simulink model "COMPONENT_MDL_Lag_QUAD_and_PEND_with_spin_rotors"  (R2021b)
settings: Solver=ode23t  StartTime=0.0  StopTime=200  FixedStep=0.001  RelTol=1e-5  EnableMultiTasking=on
undefined symbols (not defined in the file or in its folder): P_pend, P_rot, P_veh_no_props
(part 7 of 10)

== matlab function COMPONENT_MDL_Lag_QUAD_and_PEND_with_spin_rotors/bh_6DOF_and_pend/BUP/MCKGQ ==
  data: I_xx input; M output; I_xy input; I_xz input; I_yy input; I_yz input; I_zz input; Iprop_xx input; Iprop_xy input; Iprop_xz input; Iprop_yy input; Iprop_yz input; Iprop_zz input; Lx_pend input; Ly_pend input; Lz_pend input; Mbz_1 input; Mbz_2 input; Mbz_3 input; Mbz_4 input; THE_Phi input; THE_Psi input; THE_Phi_D input; THE_Psi_D input; THE_Theta input; THE_Theta_D input; THE_Phi_pend input; THE_Psi_pend input; THE_Phi_pend_D input; THE_Psi_pend_D input; THE_Theta_pend input; THE_Theta_pend_D input; Tbz_1 input; Tbz_2 input; Tbz_3 input; Tbz_4 input; Tv_Z_pend input; cg_to_mot_H input; cg_to_mot_L input; g input; m input; m_pend input; mprop input; wMOT_1 input; wMOT_2 input; wMOT_3 input; wMOT_4 input; C output; K output; G output; Q output
function [M,C,K,G,Q] = MCKGQ(I_xx,I_xy,I_xz,I_yy,I_yz,I_zz,Iprop_xx,Iprop_xy,Iprop_xz,Iprop_yy,Iprop_yz,Iprop_zz,Lx_pend,Ly_pend,Lz_pend,Mbz_1,Mbz_2,Mbz_3,Mbz_4,THE_Phi,THE_Psi,THE_Phi_D,THE_Psi_D,THE_Theta,THE_Theta_D,THE_Phi_pend,THE_Psi_pend,THE_Phi_pend_D,THE_Psi_pend_D,THE_Theta_pend,THE_Theta_pend_D,Tbz_1,Tbz_2,Tbz_3,Tbz_4,Tv_Z_pend,cg_to_mot_H,cg_to_mot_L,g,m,m_pend,mprop,wMOT_1,wMOT_2,wMOT_3,wMOT_4)
%#codegen

%    This function was generated by the Symbolic Math Toolbox version 8.6.
%    21-Sep-2020 14:08:37

M = reshape([I_xx+Iprop_xx.*4.0+(Lx_pend.^2.*m_pend)./1.2e+1+(Ly_pend.^2.*m_pend)./1.2e+1+Tv_Z_pend.^2.*m_pend+cg_to_mot_H.^2.*mprop.*4.0+cg_to_mot_L.^2.*mprop.*2.0-I_xx.*cos(THE_Theta).^2+I_yy.*cos(THE_Theta).^2-Iprop_xx.*cos(THE_Theta).^2.*4.0+Iprop_yy.*cos(THE_Theta).^2.*4.0-(Ly_pend.^2.*m_pend.*cos(THE_Theta).^2)./1.2e+1-(Ly_pend.^2.*m_pend.*cos(THE_Phi_pend).^2)./1.2e+1-(Ly_pend.^2.*m_pend.*cos(THE_Psi_pend).^2)./1.2e+1+(Lz_pend.^2.*m_pend.*cos(THE_Theta).^2)./3.0+(Lz_pend.^2.*m_pend.*cos(THE_Phi_pend).^2)./3.0+(Lz_pend.^2.*m_pend.*cos(THE_Psi_pend).^2)./3.0-I_yy.*cos(THE_Psi).^2.*cos(THE_Theta).^2+I_zz.*cos(THE_Psi).^2.*cos(THE_Theta).^2-Iprop_yy.*cos(THE_Psi).^2.*cos(THE_Theta).^2.*4.0+Iprop_zz.*cos(THE_Psi).^2.*cos(THE_Theta).^2.*4.0+I_yz.*cos(THE_Psi).*cos(THE_Theta).^2.*sin(THE_Psi).*2.0+Iprop_yz.*cos(THE_Psi).*cos(THE_Theta).^2.*sin(THE_Psi).*8.0-(Lx_pend.^2.*m_pend.*cos(THE_Psi).^2.*cos(THE_Theta).^2)./1.2e+1-(Lx_pend.^2.*m_pend.*cos(THE_Theta).^2.*cos(THE_Theta_pend).^2)./1.2e+1-(Lx_pend.^2.*m_pend.*cos(THE_Phi_pend).^2.*cos(THE_Theta_pend).^2)./1.2e+1+(Ly_pend.^2.*m_pend.*cos(THE_Psi).^2.*cos(THE_Theta).^2)./1.2e+1+(Ly_pend.^2.*m_pend.*cos(THE_Theta).^2.*cos(THE_Phi_pend).^2)./6.0+(Ly_pend.^2.*m_pend.*cos(THE_Theta).^2.*cos(THE_Psi_pend).^2)./6.0+(Ly_pend.^2.*m_pend.*cos(THE_Theta).^2.*cos(THE_Theta_pend).^2)./1.2e+1+(Ly_pend.^2.*m_pend.*cos(THE_Phi_pend).^2.*cos(THE_Psi_pend).^2)./6.0+(Ly_pend.^2.*m_pend.*cos(THE_Phi_pend).^2.*cos(THE_Theta_pend).^2)./1.2e+1-Lz_pend.^2.*m_pend.*cos(THE_Theta).^2.*cos(THE_Phi_pend).^2.*(2.0./3.0)-Lz_pend.^2.*m_pend.*cos(THE_Theta).^2.*cos(THE_Psi_pend).^2.*(2.0./3.0)-Lz_pend.^2.*m_pend.*cos(THE_Phi_pend).^2.*cos(THE_Psi_pend).^2.*(2.0./3.0)-Tv_Z_pend.^2.*m_pend.*cos(THE_Psi).^2.*cos(THE_Theta).^2-cg_to_mot_H.^2.*mprop.*cos(THE_Psi).^2.*cos(THE_Theta).^2.*4.0+cg_to_mot_L.^2.*mprop.*cos(THE_Psi).^2.*cos(THE_Theta).^2.*2.0-I_xz.*cos(THE_Psi).*cos(THE_Theta).*sin(THE_Theta).*2.0-Iprop_xz.*cos(THE_Psi).*cos(THE_Theta).*sin(THE_Theta).*8.0-I_xy.*cos(THE_Theta).*sin(THE_Psi).*sin(THE_Theta).*2.0-Iprop_xy.*cos(THE_Theta).*sin(THE_Psi).*sin(THE_Theta).*8.0+(Lx_pend.^2.*m_pend.*cos(THE_Psi).^2.*cos(THE_Theta).^2.*cos(THE_Theta_pend).^2)./6.0+(Lx_pend.^2.*m_pend.*cos(THE_Theta).^2.*cos(THE_Phi_pend).^2.*cos(THE_Theta_pend).^2)./6.0-(Ly_pend.^2.*m_pend.*cos(THE_Psi).^2.*cos(THE_Theta).^2.*cos(THE_Phi_pend).^2)./1.2e+1-(Ly_pend.^2.*m_pend.*cos(THE_Psi).^2.*cos(THE_Theta).^2.*cos(THE_Psi_pend).^2)./1.2e+1-(Ly_pend.^2.*m_pend.*cos(THE_Psi).^2.*cos(THE_Theta).^2.*cos(THE_Theta_pend).^2)./6.0-(Ly_pend.^2.*m_pend.*cos(THE_Theta).^2.*cos(THE_Phi_pend).^2.*cos(THE_Psi_pend).^2)./3.0-(Ly_pend.^2.*m_pend.*cos(THE_Theta).^2.*cos(THE_Phi_pend).^2.*cos(THE_Theta_pend).^2)./6.0-(Ly_pend.^2.*m_pend.*cos(THE_Theta).^2.*cos(THE_Psi_pend).^2.*cos(THE_Theta_pend).^2)./1.2e+1-(Ly_pend.^2.*m_pend.*cos(THE_Phi_pend).^2.*cos(THE_Psi_pend).^2.*cos(THE_Theta_pend).^2)./1.2e+1+(Lz_pend.^2.*m_pend.*cos(THE_Psi).^2.*cos(THE_Theta).^2.*cos(THE_Phi_pend).^2)./3.0+(Lz_pend.^2.*m_pend.*cos(THE_Psi).^2.*cos(THE_Theta).^2.*cos(THE_Psi_pend).^2)./3.0+Lz_pend.^2.*m_pend.*cos(THE_Theta).^2.*cos(THE_Phi_pend).^2.*cos(THE_Psi_pend).^2.*(4.0./3.0)+(Lz_pend.^2.*m_pend.*cos(THE_Theta).^2.*cos(THE_Psi_pend).^2.*cos(THE_Theta_pend).^2)./3.0+(Lz_pend.^2.*m_pend.*cos(THE_Phi_pend).^2.*cos(THE_Psi_pend).^2.*cos(THE_Theta_pend).^2)./3.0+Lz_pend.*Tv_Z_pend.*m_pend.*cos(THE_Psi_pend).*cos(THE_Theta_pend)-(Lx_pend.^2.*m_pend.*cos(THE_Psi).^2.*cos(THE_Theta).^2.*cos(THE_Phi_pend).^2.*cos(THE_Theta_pend).^2)./1.2e+1+(Ly_pend.^2.*m_pend.*cos(THE_Psi).^2.*cos(THE_Theta).^2.*cos(THE_Phi_pend).^2.*cos(THE_Psi_pend).^2)./6.0+(Ly_pend.^2.*m_pend.*cos(THE_Psi).^2.*cos(THE_Theta).^2.*cos(THE_Phi_pend).^2.*cos(THE_Theta_pend).^2)./1.2e+1+(Ly_pend.^2.*m_pend.*cos(THE_Psi).^2.*cos(THE_Theta).^2.*cos(THE_Psi_pend).^2.*cos(THE_Theta_pend).^2)./6.0+(Ly_pend.^2.*m_pend.*cos(THE_Theta).^2.*cos(THE_Phi_pend).^2.*cos(THE_Psi_pend).^2.*cos(THE_Theta_pend).^2)./6.0-Lz_pend.^2.*m_pend.*cos(THE_Psi).^2.*cos(THE_Theta).^2.*cos(THE_Phi_pend).^2.*cos(THE_Psi_pend).^2.*(2.0./3.0)-Lz_pend.^2.*m_pend.*cos(THE_Psi).^2.*cos(THE_Theta).^2.*cos(THE_Psi_pend).^2.*cos(THE_Theta_pend).^2.*(2.0./3.0)-Lz_pend.^2.*m_pend.*cos(THE_Theta).^2.*cos(THE_Phi_pend).^2.*cos(THE_Psi_pend).^2.*cos(THE_Theta_pend).^2.*(2.0./3.0)-Lz_pend.*Tv_Z_pend.*m_pend.*cos(THE_Psi).^2.*cos(THE_Theta).^2.*cos(THE_Psi_pend).*cos(THE_Theta_pend)+(Ly_pend.^2.*m_pend.*cos(THE_Theta).*cos(THE_Phi_pend).*sin(THE_Psi).*sin(THE_Theta).*sin(THE_Phi_pend))./6.0+(Ly_pend.^2.*m_pend.*cos(THE_Phi_pend).*cos(THE_Psi_pend).*sin(THE_Phi_pend).*sin(THE_Psi_pend).*sin(THE_Theta_pend))./6.0-Lz_pend.^2.*m_pend.*cos(THE_Theta).*cos(THE_Phi_pend).*sin(THE_Psi).*sin(THE_Theta).*sin(THE_Phi_pend).*(2.0./3.0)-Lz_pend.^2.*m_pend.*cos(THE_Phi_pend).*cos(THE_Psi_pend).*sin(THE_Phi_pend).*sin(THE_Psi_pend).*sin(THE_Theta_pend).*(2.0./3.0)-(Ly_pend.^2.*m_pend.*cos(THE_Psi).^2.*cos(THE_Theta).^2.*cos(THE_Phi_pend).^2.*cos(THE_Psi_pend).^2.*cos(THE_Theta_pend).^2)./1.2e+1+(Lz_pend.^2.*m_pend.*cos(THE_Psi).^2.*cos(THE_Theta).^2.*cos(THE_Phi_pend).^2.*cos(THE_Psi_pend).^2.*cos(THE_Theta_pend).^2)./3.0-(Ly_pend.^2.*m_pend.*cos(THE_Theta).*cos(THE_Psi_pend).*sin(THE_Psi).*sin(THE_Theta).*sin(THE_Psi_pend).*sin(THE_Theta_pend))./6.0+Lz_pend.^2.*m_pend.*cos(THE_Theta).*cos(THE_Psi_pend).*sin(THE_Psi).*sin(THE_Theta).*sin(THE_Psi_pend).*sin(THE_Theta_pend).*(2.0./3.0)+Lz_pend.*Tv_Z_pend.*m_pend.*cos(THE_Psi).*cos(THE_Theta).*sin(THE_Theta).*sin(THE_Phi_pend).*sin(THE_Psi_pend)+(Lx_pend.^2.*m_pend.*cos(THE_Theta).*cos(THE_Phi_pend).*cos(THE_Theta_pend).^2.*sin(THE_Psi).*sin(THE_Theta).*sin(THE_Phi_pend))./6.0+(Lx_pend.^2.*m_pend.*cos(THE_Psi).*cos(THE_Theta).^2.*cos(THE_Theta_pend).*sin(THE_Psi).*sin(THE_Phi_pend).*sin(THE_Theta_pend))./6.0-(Ly_pend.^2.*m_pend.*cos(THE_Theta).*cos(THE_Phi_pend).*cos(THE_Psi_pend).^2.*sin(THE_Psi).*sin(THE_Theta).*sin(THE_Phi_pend))./3.0-(Ly_pend.^2.*m_pend.*cos(THE_Theta).*cos(THE_Phi_pend).*cos(THE_Theta_pend).^2.*sin(THE_Psi).*sin(THE_Theta).*sin(THE_Phi_pend))./6.0-(Ly_pend.^2.*m_pend.*cos(THE_Psi).*cos(THE_Theta).^2.*cos(THE_Theta_pend).*sin(THE_Psi).*sin(THE_Phi_pend).*sin(THE_Theta_pend))./6.0-(Ly_pend.^2.*m_pend.*cos(THE_Theta).^2.*cos(THE_Phi_pend).*cos(THE_Psi_pend).*sin(THE_Phi_pend).*sin(THE_Psi_pend).*sin(THE_Theta_pend))./3.0+Lz_pend.^2.*m_pend.*cos(THE_Theta).*cos(THE_Phi_pend).*cos(THE_Psi_pend).^2.*sin(THE_Psi).*sin(THE_Theta).*sin(THE_Phi_pend).*(4.0./3.0)+Lz_pend.^2.*m_pend.*cos(THE_Theta).^2.*cos(THE_Phi_pend).*cos(THE_Psi_pend).*sin(THE_Phi_pend).*sin(THE_Psi_pend).*sin(THE_Theta_pend).*(4.0./3.0)+Lz_pend.*Tv_Z_pend.*m_pend.*cos(THE_Psi).*cos(THE_Theta).^2.*cos(THE_Phi_pend).*sin(THE_Psi).*sin(THE_Psi_pend)-(Lx_pend.^2.*m_pend.*cos(THE_Psi).*cos(THE_Theta).*cos(THE_Phi_pend).*cos(THE_Theta_pend).*sin(THE_Theta).*sin(THE_Theta_pend))./6.0+(Ly_pend.^2.*m_pend.*cos(THE_Psi).*cos(THE_Theta).*cos(THE_Phi_pend).*cos(THE_Theta_pend).*sin(THE_Theta).*sin(THE_Theta_pend))./6.0+(Ly_pend.^2.*m_pend.*cos(THE_Theta).*cos(THE_Phi_pend).^2.*cos(THE_Psi_pend).*sin(THE_Psi).*sin(THE_Theta).*sin(THE_Psi_pend).*sin(THE_Theta_pend))./3.0-Lz_pend.^2.*m_pend.*cos(THE_Theta).*cos(THE_Phi_pend).^2.*cos(THE_Psi_pend).*sin(THE_Psi).*sin(THE_Theta).*sin(THE_Psi_pend).*sin(THE_Theta_pend).*(4.0./3.0)-Lz_pend.*Tv_Z_pend.*m_pend.*cos(THE_Psi).*cos(THE_Theta).^2.*cos(THE_Psi_pend).*sin(THE_Psi).*sin(THE_Phi_pend).*sin(THE_Theta_pend)+(Ly_pend.^2.*m_pend.*cos(THE_Theta).*cos(THE_Phi_pend).*cos(THE_Psi_pend).^2.*cos(THE_Theta_pend).^2.*sin(THE_Psi).*sin(THE_Theta).*sin(THE_Phi_pend))./6.0+(Ly_pend.^2.*m_pend.*cos(THE_Psi).*cos(THE_Theta).^2.*cos(THE_Psi_pend).^2.*cos(THE_Theta_pend).*sin(THE_Psi).*sin(THE_Phi_pend).*sin(THE_Theta_pend))./6.0+(Ly_pend.^2.*m_pend.*cos(THE_Psi).^2.*cos(THE_Theta).^2.*cos(THE_Phi_pend).*cos(THE_Psi_pend).*sin(THE_Phi_pend).*sin(THE_Psi_pend).*sin(THE_Theta_pend))./6.0-Lz_pend.^2.*m_pend.*cos(THE_Theta).*cos(THE_Phi_pend).*cos(THE_Psi_pend).^2.*cos(THE_Theta_pend).^2.*sin(THE_Psi).*sin(THE_Theta).*sin(THE_Phi_pend).*(2.0./3.0)-Lz_pend.^2.*m_pend.*cos(THE_Psi).*cos(THE_Theta).^2.*cos(THE_Psi_pend).^2.*cos(THE_Theta_pend).*sin(THE_Psi).*sin(THE_Phi_pend).*sin(THE_Theta_pend).*(2.0./3.0)-Lz_pend.^2.*m_pend.*cos(THE_Psi).^2.*cos(THE_Theta).^2.*cos(THE_Phi_pend).*cos(THE_Psi_pend).*sin(THE_Phi_pend).*sin(THE_Psi_pend).*sin(THE_Theta_pend).*(2.0./3.0)-(Ly_pend.^2.*m_pend.*cos(THE_Psi).*cos(THE_Theta).*cos(THE_Psi_pend).*cos(THE_Theta_pend).*sin(THE_Theta).*sin(THE_Phi_pend).*sin(THE_Psi_pend))./6.0+Lz_pend.^2.*m_pend.*cos(THE_Psi).*cos(THE_Theta).*cos(THE_Psi_pend).*cos(THE_Theta_pend).*sin(THE_Theta).*sin(THE_Phi_pend).*sin(THE_Psi_pend).*(2.0./3.0)+Lz_pend.*Tv_Z_pend.*m_pend.*cos(THE_Psi).*cos(THE_Theta).*cos(THE_Phi_pend).*cos(THE_Psi_pend).*sin(THE_Theta).*sin(THE_Theta_pend)-(Ly_pend.^2.*m_pend.*cos(THE_Psi).*cos(THE_Theta).^2.*cos(THE_Phi_pend).*cos(THE_Psi_pend).*cos(THE_Theta_pend).*sin(THE_Psi).*sin(THE_Psi_pend))./6.0-(Ly_pend.^2.*m_pend.*cos(THE_Psi).*cos(THE_Theta).*cos(THE_Phi_pend).*cos(THE_Psi_pend).^2.*cos(THE_Theta_pend).*sin(THE_Theta).*sin(THE_Theta_pend))./6.0+Lz_pend.^2.*m_pend.*cos(THE_Psi).*cos(THE_Theta).^2.*cos(THE_Phi_pend).*cos(THE_Psi_pend).*cos(THE_Theta_pend).*sin(THE_Psi).*sin(THE_Psi_pend).*(2.0./3.0)+Lz_pend.^2.*m_pend.*cos(THE_Psi).*cos(THE_Theta).*cos(THE_Phi_pend).*cos(THE_Psi_pend).^2.*cos(THE_Theta_pend).*sin(THE_Theta).*sin(THE_Theta_pend).*(2.0./3.0),-I_yz.*cos(THE_Theta)-Iprop_yz.*cos(THE_Theta).*4.0-I_xy.*cos(THE_Psi).*sin(THE_Theta)-Iprop_xy.*cos(THE_Psi).*sin(THE_Theta).*4.0+I_xz.*sin(THE_Psi).*sin(THE_Theta)+Iprop_xz.*sin(THE_Psi).*sin(THE_Theta).*4.0+I_yz.*cos(THE_Psi).^2.*cos(THE_Theta).*2.0+Iprop_yz.*cos(THE_Psi).^2.*cos(THE_Theta).*8.0+I_yy.*cos(THE_Psi).*cos(THE_Theta).*sin(THE_Psi)-I_zz.*cos(THE_Psi).*cos(THE_Theta).*sin(THE_Psi)+Iprop_yy.*cos(THE_Psi).*cos(THE_Theta).*sin(THE_Psi).*4.0-Iprop_zz.*cos(THE_Psi).*cos(THE_Theta).*sin(THE_Psi).*4.0+(Lx_pend.^2.*m_pend.*cos(THE_Psi).*cos(THE_Theta).*sin(THE_Psi))./1.2e+1-(Ly_pend.^2.*m_pend.*cos(THE_Psi).*cos(THE_Theta).*sin(THE_Psi))./1.2e+1+Tv_Z_pend.^2.*m_pend.*cos(THE_Psi).*cos(THE_Theta).*sin(THE_Psi)+cg_to_mot_H.^2.*mprop.*cos(THE_Psi).*cos(THE_Theta).*sin(THE_Psi).*4.0-cg_to_mot_L.^2.*mprop.*cos(THE_Psi).*cos(THE_Theta).*sin(THE_Psi).*2.0-(Lx_pend.^2.*m_pend.*cos(THE_Theta).*cos(THE_Theta_pend).*sin(THE_Phi_pend).*sin(THE_Theta_pend))./1.2e+1+(Ly_pend.^2.*m_pend.*cos(THE_Psi).*cos(THE_Phi_pend).*sin(THE_Theta).*sin(THE_Phi_pend))./1.2e+1+(Ly_pend.^2.*m_pend.*cos(THE_Theta).*cos(THE_Theta_pend).*sin(THE_Phi_pend).*sin(THE_Theta_pend))./1.2e+1-(Lz_pend.^2.*m_pend.*cos(THE_Psi).*cos(THE_Phi_pend).*sin(THE_Theta).*sin(THE_Phi_pend))./3.0-(Lz_pend.*Tv_Z_pend.*m_pend.*cos(THE_Theta).*cos(THE_Phi_pend).*sin(THE_Psi_pend))./2.0-(Lx_pend.^2.*m_pend.*cos(THE_Psi).*cos(THE_Theta).*cos(THE_Theta_pend).^2.*sin(THE_Psi))./6.0+(Ly_pend.^2.*m_pend.*cos(THE_Psi).*cos(THE_Theta).*cos(THE_Phi_pend).^2.*sin(THE_Psi))./1.2e+1+(Ly_pend.^2.*m_pend.*cos(THE_Psi).*cos(THE_Theta).*cos(THE_Psi_pend).^2.*sin(THE_Psi))./1.2e+1+(Ly_pend.^2.*m_pend.*cos(THE_Psi).*cos(THE_Theta).*cos(THE_Theta_pend).^2.*sin(THE_Psi))./6.0-(Lz_pend.^2.*m_pend.*cos(THE_Psi).*cos(THE_Theta).*cos(THE_Phi_pend).^2.*sin(THE_Psi))./3.0-(Lz_pend.^2.*m_pend.*cos(THE_Psi).*cos(THE_Theta).*cos(THE_Psi_pend).^2.*sin(THE_Psi))./3.0+(Ly_pend.^2.*m_pend.*cos(THE_Theta).*cos(THE_Phi_pend).*cos(THE_Psi_pend).*cos(THE_Theta_pend).*sin(THE_Psi_pend))./1.2e+1-(Lz_pend.^2.*m_pend.*cos(THE_Theta).*cos(THE_Phi_pend).*cos(THE_Psi_pend).*cos(THE_Theta_pend).*sin(THE_Psi_pend))./3.0+(Lx_pend.^2.*m_pend.*cos(THE_Phi_pend).*cos(THE_Theta_pend).*sin(THE_Psi).*sin(THE_Theta).*sin(THE_Theta_pend))./1.2e+1-(Ly_pend.^2.*m_pend.*cos(THE_Psi).*cos(THE_Psi_pend).*sin(THE_Theta).*sin(THE_Psi_pend).*sin(THE_Theta_pend))./1.2e+1-(Ly_pend.^2.*m_pend.*cos(THE_Phi_pend).*cos(THE_Theta_pend).*sin(THE_Psi).*sin(THE_Theta).*sin(THE_Theta_pend))./1.2e+1+(Lz_pend.^2.*m_pend.*cos(THE_Psi).*cos(THE_Psi_pend).*sin(THE_Theta).*sin(THE_Psi_pend).*sin(THE_Theta_pend))./3.0+(Lz_pend.*Tv_Z_pend.*m_pend.*cos(THE_Theta).*cos(THE_Psi_pend).*sin(THE_Phi_pend).*sin(THE_Theta_pend))./2.0-(Lz_pend.*Tv_Z_pend.*m_pend.*sin(THE_Psi).*sin(THE_Theta).*sin(THE_Phi_pend).*sin(THE_Psi_pend))./2.0+(Lx_pend.^2.*m_pend.*cos(THE_Psi).*cos(THE_Phi_pend).*cos(THE_Theta_pend).^2.*sin(THE_Theta).*sin(THE_Phi_pend))./1.2e+1+(Lx_pend.^2.*m_pend.*cos(THE_Psi).^2.*cos(THE_Theta).*cos(THE_Theta_pend).*sin(THE_Phi_pend).*sin(THE_Theta_pend))./6.0-(Ly_pend.^2.*m_pend.*cos(THE_Psi).*cos(THE_Phi_pend).*cos(THE_Psi_pend).^2.*sin(THE_Theta).*sin(THE_Phi_pend))./6.0-(Ly_pend.^2.*m_pend.*cos(THE_Psi).*cos(THE_Phi_pend).*cos(THE_Theta_pend).^2.*sin(THE_Theta).*sin(THE_Phi_pend))./1.2e+1-(Ly_pend.^2.*m_pend.*cos(THE_Psi).^2.*cos(THE_Theta).*cos(THE_Theta_pend).*sin(THE_Phi_pend).*sin(THE_Theta_pend))./6.0-(Ly_pend.^2.*m_pend.*cos(THE_Theta).*cos(THE_Psi_pend).^2.*cos(THE_Theta_pend).*sin(THE_Phi_pend).*sin(THE_Theta_pend))./1.2e+1+Lz_pend.^2.*m_pend.*cos(THE_Psi).*cos(THE_Phi_pend).*cos(THE_Psi_pend).^2.*sin(THE_Theta).*sin(THE_Phi_pend).*(2.0./3.0)+(Lz_pend.^2.*m_pend.*cos(THE_Theta).*cos(THE_Psi_pend).^2.*cos(THE_Theta_pend).*sin(THE_Phi_pend).*sin(THE_Theta_pend))./3.0+Lz_pend.*Tv_Z_pend.*m_pend.*cos(THE_Psi).^2.*cos(THE_Theta).*cos(THE_Phi_pend).*sin(THE_Psi_pend)+(Lx_pend.^2.*m_pend.*cos(THE_Psi).*cos(THE_Theta).*cos(THE_Phi_pend).^2.*cos(THE_Theta_pend).^2.*sin(THE_Psi))./1.2e+1-(Ly_pend.^2.*m_pend.*cos(THE_Psi).*cos(THE_Theta).*cos(THE_Phi_pend).^2.*cos(THE_Psi_pend).^2.*sin(THE_Psi))./6.0-(Ly_pend.^2.*m_pend.*cos(THE_Psi).*cos(THE_Theta).*cos(THE_Phi_pend).^2.*cos(THE_Theta_pend).^2.*sin(THE_Psi))./1.2e+1-(Ly_pend.^2.*m_pend.*cos(THE_Psi).*cos(THE_Theta).*cos(THE_Psi_pend).^2.*cos(THE_Theta_pend).^2.*sin(THE_Psi))./6.0+Lz_pend.^2.*m_pend.*cos(THE_Psi).*cos(THE_Theta).*cos(THE_Phi_pend).^2.*cos(THE_Psi_pend).^2.*sin(THE_Psi).*(2.0./3.0)+Lz_pend.^2.*m_pend.*cos(THE_Psi).*cos(THE_Theta).*cos(THE_Psi_pend).^2.*cos(THE_Theta_pend).^2.*sin(THE_Psi).*(2.0./3.0)+(Ly_pend.^2.*m_pend.*cos(THE_Psi_pend).*cos(THE_Theta_pend).*sin(THE_Psi).*sin(THE_Theta).*sin(THE_Phi_pend).*sin(THE_Psi_pend))./1.2e+1-(Lz_pend.^2.*m_pend.*cos(THE_Psi_pend).*cos(THE_Theta_pend).*sin(THE_Psi).*sin(THE_Theta).*sin(THE_Phi_pend).*sin(THE_Psi_pend))./3.0+Lz_pend.*Tv_Z_pend.*m_pend.*cos(THE_Psi).*cos(THE_Theta).*cos(THE_Psi_pend).*cos(THE_Theta_pend).*sin(THE_Psi)-(Lz_pend.*Tv_Z_pend.*m_pend.*cos(THE_Phi_pend).*cos(THE_Psi_pend).*sin(THE_Psi).*sin(THE_Theta).*sin(THE_Theta_pend))./2.0-(Ly_pend.^2.*m_pend.*cos(THE_Psi).^2.*cos(THE_Theta).*cos(THE_Phi_pend).*cos(THE_Psi_pend).*cos(THE_Theta_pend).*sin(THE_Psi_pend))./6.0+Lz_pend.^2.*m_pend.*cos(THE_Psi).^2.*cos(THE_Theta).*cos(THE_Phi_pend).*cos(THE_Psi_pend).*cos(THE_Theta_pend).*sin(THE_Psi_pend).*(2.0./3.0)+(Ly_pend.^2.*m_pend.*cos(THE_Psi).*cos(THE_Phi_pend).^2.*cos(THE_Psi_pend).*sin(THE_Theta).*sin(THE_Psi_pend).*sin(THE_Theta_pend))./6.0+(Ly_pend.^2.*m_pend.*cos(THE_Phi_pend).*cos(THE_Psi_pend).^2.*cos(THE_Theta_pend).*sin(THE_Psi).*sin(THE_Theta).*sin(THE_Theta_pend))./1.2e+1-Lz_pend.^2.*m_pend.*cos(THE_Psi).*cos(THE_Phi_pend).^2.*cos(THE_Psi_pend).*sin(THE_Theta).*sin(THE_Psi_pend).*sin(THE_Theta_pend).*(2.0./3.0)-(Lz_pend.^2.*m_pend.*cos(THE_Phi_pend).*cos(THE_Psi_pend).^2.*cos(THE_Theta_pend).*sin(THE_Psi).*sin(THE_Theta).*sin(THE_Theta_pend))./3.0-Lz_pend.*Tv_Z_pend.*m_pend.*cos(THE_Psi).^2.*cos(THE_Theta).*cos(THE_Psi_pend).*sin(THE_Phi_pend).*sin(THE_Theta_pend)+(Ly_pend.^2.*m_pend.*cos(THE_Psi).*cos(THE_Phi_pend).*cos(THE_Psi_pend).^2.*cos(THE_Theta_pend).^2.*sin(THE_Theta).*sin(THE_Phi_pend))./1.2e+1+(Ly_pend.^2.*m_pend.*cos(THE_Psi).^2.*cos(THE_Theta).*cos(THE_Psi_pend).^2.*cos(THE_Theta_pend).*sin(THE_Phi_pend).*sin(THE_Theta_pend))./6.0-(Lz_pend.^2.*m_pend.*cos(THE_Psi).*cos(THE_Phi_pend).*cos(THE_Psi_pend).^2.*cos(THE_Theta_pend).^2.*sin(THE_Theta).*sin(THE_Phi_pend))./3.0-Lz_pend.^2.*m_pend.*cos(THE_Psi).^2.*cos(THE_Theta).*cos(THE_Psi_pend).^2.*cos(THE_Theta_pend).*sin(THE_Phi_pend).*sin(THE_Theta_pend).*(2.0./3.0)+(Ly_pend.^2.*m_pend.*cos(THE_Psi).*cos(THE_Theta).*cos(THE_Phi_pend).^2.*cos(THE_Psi_pend).^2.*cos(THE_Theta_pend).^2.*sin(THE_Psi))./1.2e+1-(Lz_pend.^2.*m_pend.*cos(THE_Psi).*cos(THE_Theta).*cos(THE_Phi_pend).^2.*cos(THE_Psi_pend).^2.*cos(THE_Theta_pend).^2.*sin(THE_Psi))./3.0-(Ly_pend.^2.*m_pend.*cos(THE_Psi).*cos(THE_Theta).*cos(THE_Phi_pend).*cos(THE_Psi_pend).*sin(THE_Psi).*sin(THE_Phi_pend).*sin(THE_Psi_pend).*sin(THE_Theta_pend))./6.0+Lz_pend.^2.*m_pend.*cos(THE_Psi).*cos(THE_Theta).*cos(THE_Phi_pend).*cos(THE_Psi_pend).*sin(THE_Psi).*sin(THE_Phi_pend).*sin(THE_Psi_pend).*sin(THE_Theta_pend).*(2.0./3.0),-I_xx.*sin(THE_Theta)-Iprop_xx.*sin(THE_Theta).*4.0+I_xz.*cos(THE_Psi).*cos(THE_Theta)+Iprop_xz.*cos(THE_Psi).*cos(THE_Theta).*4.0+I_xy.*cos(THE_Theta).*sin(THE_Psi)+Iprop_xy.*cos(THE_Theta).*sin(THE_Psi).*4.0-(Lx_pend.^2.*m_pend.*sin(THE_Theta))./1.2e+1-(Ly_pend.^2.*m_pend.*sin(THE_Theta))./1.2e+1-Tv_Z_pend.^2.*m_pend.*sin(THE_Theta)-cg_to_mot_H.^2.*mprop.*sin(THE_Theta).*4.0-cg_to_mot_L.^2.*mprop.*sin(THE_Theta).*2.0+(Ly_pend.^2.*m_pend.*cos(THE_Phi_pend).^2.*sin(THE_Theta))./1.2e+1+(Ly_pend.^2.*m_pend.*cos(THE_Psi_pend).^2.*sin(THE_Theta))./1.2e+1-(Lz_pend.^2.*m_pend.*cos(THE_Phi_pend).^2.*sin(THE_Theta))./3.0-(Lz_pend.^2.*m_pend.*cos(THE_Psi_pend).^2.*sin(THE_Theta))./3.0+(Lx_pend.^2.*m_pend.*cos(THE_Phi_pend).^2.*cos(THE_Theta_pend).^2.*sin(THE_Theta))./1.2e+1-(Ly_pend.^2.*m_pend.*cos(THE_Phi_pend).^2.*cos(THE_Psi_pend).^2.*sin(THE_Theta))./6.0-(Ly_pend.^2.*m_pend.*cos(THE_Phi_pend).^2.*cos(THE_Theta_pend).^2.*sin(THE_Theta))./1.2e+1+Lz_pend.^2.*m_pend.*cos(THE_Phi_pend).^2.*cos(THE_Psi_pend).^2.*sin(THE_Theta).*(2.0./3.0)-(Ly_pend.^2.*m_pend.*cos(THE_Theta).*cos(THE_Phi_pend).*sin(THE_Psi).*sin(THE_Phi_pend))./1.2e+1+(Lz_pend.^2.*m_pend.*cos(THE_Theta).*cos(THE_Phi_pend).*sin(THE_Psi).*sin(THE_Phi_pend))./3.0+(Ly_pend.^2.*m_pend.*cos(THE_Phi_pend).^2.*cos(THE_Psi_pend).^2.*cos(THE_Theta_pend).^2.*sin(THE_Theta))./1.2e+1-(Lz_pend.^2.*m_pend.*cos(THE_Phi_pend).^2.*cos(THE_Psi_pend).^2.*cos(THE_Theta_pend).^2.*sin(THE_Theta))./3.0-Lz_pend.*Tv_Z_pend.*m_pend.*cos(THE_Psi_pend).*cos(THE_Theta_pend).*sin(THE_Theta)+(Lx_pend.^2.*m_pend.*cos(THE_Psi).*cos(THE_Theta).*cos(THE_Phi_pend).*cos(THE_Theta_pend).*sin(THE_Theta_pend))./1.2e+1-(Ly_pend.^2.*m_pend.*cos(THE_Psi).*cos(THE_Theta).*cos(THE_Phi_pend).*cos(THE_Theta_pend).*sin(THE_Theta_pend))./1.2e+1+(Ly_pend.^2.*m_pend.*cos(THE_Theta).*cos(THE_Psi_pend).*sin(THE_Psi).*sin(THE_Psi_pend).*sin(THE_Theta_pend))./1.2e+1-(Lz_pend.^2.*m_pend.*cos(THE_Theta).*cos(THE_Psi_pend).*sin(THE_Psi).*sin(THE_Psi_pend).*sin(THE_Theta_pend))./3.0-(Lz_pend.*Tv_Z_pend.*m_pend.*cos(THE_Psi).*cos(THE_Theta).*sin(THE_Phi_pend).*sin(THE_Psi_pend))./2.0-(Lx_pend.^2.*m_pend.*cos(THE_Theta).*cos(THE_Phi_pend).*cos(THE_Theta_pend).^2.*sin(THE_Psi).*sin(THE_Phi_pend))./1.2e+1+(Ly_pend.^2.*m_pend.*cos(THE_Theta).*cos(THE_Phi_pend).*cos(THE_Psi_pend).^2.*sin(THE_Psi).*sin(THE_Phi_pend))./6.0+(Ly_pend.^2.*m_pend.*cos(THE_Theta).*cos(THE_Phi_pend).*cos(THE_Theta_pend).^2.*sin(THE_Psi).*sin(THE_Phi_pend))./1.2e+1-Lz_pend.^2.*m_pend.*cos(THE_Theta).*cos(THE_Phi_pend).*cos(THE_Psi_pend).^2.*sin(THE_Psi).*sin(THE_Phi_pend).*(2.0./3.0)-(Ly_pend.^2.*m_pend.*cos(THE_Phi_pend).*cos(THE_Psi_pend).*sin(THE_Theta).*sin(THE_Phi_pend).*sin(THE_Psi_pend).*sin(THE_Theta_pend))./6.0+Lz_pend.^2.*m_pend.*cos(THE_Phi_pend).*cos(THE_Psi_pend).*sin(THE_Theta).*sin(THE_Phi_pend).*sin(THE_Psi_pend).*sin(THE_Theta_pend).*(2.0./3.0)-(Lz_pend.*Tv_Z_pend.*m_pend.*cos(THE_Psi).*cos(THE_Theta).*cos(THE_Phi_pend).*cos(THE_Psi_pend).*sin(THE_Theta_pend))./2.0+(Ly_pend.^2.*m_pend.*cos(THE_Psi).*cos(THE_Theta).*cos(THE_Phi_pend).*cos(THE_Psi_pend).^2.*cos(THE_Theta_pend).*sin(THE_Theta_pend))./1.2e+1-(Lz_pend.^2.*m_pend.*cos(THE_Psi).*cos(THE_Theta).*cos(THE_Phi_pend).*cos(THE_Psi_pend).^2.*cos(THE_Theta_pend).*sin(THE_Theta_pend))./3.0-(Ly_pend.^2.*m_pend.*cos(THE_Theta).*cos(THE_Phi_pend).^2.*cos(THE_Psi_pend).*sin(THE_Psi).*sin(THE_Psi_pend).*sin(THE_Theta_pend))./6.0+Lz_pend.^2.*m_pend.*cos(THE_Theta).*cos(THE_Phi_pend).^2.*cos(THE_Psi_pend).*sin(THE_Psi).*sin(THE_Psi_pend).*sin(THE_Theta_pend).*(2.0./3.0)-(Ly_pend.^2.*m_pend.*cos(THE_Theta).*cos(THE_Phi_pend).*cos(THE_Psi_pend).^2.*cos(THE_Theta_pend).^2.*sin(THE_Psi).*sin(THE_Phi_pend))./1.2e+1+(Lz_pend.^2.*m_pend.*cos(THE_Theta).*cos(THE_Phi_pend).*cos(THE_Psi_pend).^2.*cos(THE_Theta_pend).^2.*sin(THE_Psi).*sin(THE_Phi_pend))./3.0+(Ly_pend.^2.*m_pend.*cos(THE_Psi).*cos(THE_Theta).*cos(THE_Psi_pend).*cos(THE_Theta_pend).*sin(THE_Phi_pend).*sin(THE_Psi_pend))./1.2e+1-(Lz_pend.^2.*m_pend.*cos(THE_Psi).*cos(THE_Theta).*cos(THE_Psi_pend).*cos(THE_Theta_pend).*sin(THE_Phi_pend).*sin(THE_Psi_pend))./3.0,Tv_Z_pend.*m_pend.*cos(THE_Phi).*sin(THE_Psi)+cg_to_mot_H.*mprop.*cos(THE_Phi).*sin(THE_Psi).*4.0-Tv_Z_pend.*m_pend.*cos(THE_Psi).*sin(THE_Phi).*sin(THE_Theta)-cg_to_mot_H.*mprop.*cos(THE_Psi).*sin(THE_Phi).*sin(THE_Theta).*4.0+(Lz_pend.*m_pend.*cos(THE_Phi).*cos(THE_Psi).*cos(THE_Phi_pend).*sin(THE_Psi_pend))./2.0+(Lz_pend.*m_pend.*cos(THE_Phi).*cos(THE_Psi_pend).*cos(THE_Theta_pend).*sin(THE_Psi))./2.0-(Lz_pend.*m_pend.*cos(THE_Theta).*sin(THE_Phi).*sin(THE_Phi_pend).*sin(THE_Psi_pend))./2.0-(Lz_pend.*m_pend.*cos(THE_Psi).*cos(THE_Psi_pend).*cos(THE_Theta_pend).*sin(THE_Phi).*sin(THE_Theta))./2.0-(Lz_pend.*m_pend.*cos(THE_Phi).*cos(THE_Psi).*cos(THE_Psi_pend).*sin(THE_Phi_pend).*sin(THE_Theta_pend))./2.0-(Lz_pend.*m_pend.*cos(THE_Theta).*cos(THE_Phi_pend).*cos(THE_Psi_pend).*sin(THE_Phi).*sin(THE_Theta_pend))./2.0+(Lz_pend.*m_pend.*cos(THE_Phi_pend).*sin(THE_Phi).*sin(THE_Psi).*sin(THE_Theta).*sin(THE_Psi_pend))./2.0-(Lz_pend.*m_pend.*cos(THE_Psi_pend).*sin(THE_Phi).*sin(THE_Psi).*sin(THE_Theta).*sin(THE_Phi_pend).*sin(THE_Theta_pend))./2.0,Tv_Z_pend.*m_pend.*sin(THE_Phi).*sin(THE_Psi)+cg_to_mot_H.*mprop.*sin(THE_Phi).*sin(THE_Psi).*4.0+Tv_Z_pend.*m_pend.*cos(THE_Phi).*cos(THE_Psi).*sin(THE_Theta)+cg_to_mot_H.*mprop.*cos(THE_Phi).*cos(THE_Psi).*sin(THE_Theta).*4.0+(Lz_pend.*m_pend.*cos(THE_Psi).*cos(THE_Phi_pend).*sin(THE_Phi).*sin(THE_Psi_pend))./2.0+(Lz_pend.*m_pend.*cos(THE_Phi).*cos(THE_Theta).*sin(THE_Phi_pend).*sin(THE_Psi_pend))./2.0+(Lz_pend.*m_pend.*cos(THE_Psi_pend).*cos(THE_Theta_pend).*sin(THE_Phi).*sin(THE_Psi))./2.0+(Lz_pend.*m_pend.*cos(THE_Phi).*cos(THE_Psi).*cos(THE_Psi_pend).*cos(THE_Theta_pend).*sin(THE_Theta))./2.0+(Lz_pend.*m_pend.*cos(THE_Phi).*cos(THE_Theta).*cos(THE_Phi_pend).*cos(THE_Psi_pend).*sin(THE_Theta_pend))./2.0-(Lz_pend.*m_pend.*cos(THE_Phi).*cos(THE_Phi_pend).*sin(THE_Psi).*sin(THE_Theta).*sin(THE_Psi_pend))./2.0-(Lz_pend.*m_pend.*cos(THE_Psi).*cos(THE_Psi_pend).*sin(THE_Phi).*sin(THE_Phi_pend).*sin(THE_Theta_pend))./2.0+(Lz_pend.*m_pend.*cos(THE_Phi).*cos(THE_Psi_pend).*sin(THE_Psi).*sin(THE_Theta).*sin(THE_Phi_pend).*sin(THE_Theta_pend))./2.0,0.0,(Ly_pend.^2.*m_pend.*cos(THE_Psi).*cos(THE_Theta))./1.2e+1+(Lz_pend.^2.*m_pend.*cos(THE_Psi).*cos(THE_Theta))./3.0+(Lx_pend.^2.*m_pend.*cos(THE_Psi).*cos(THE_Theta).*cos(THE_Theta_pend).^2)./1.2e+1-(Ly_pend.^2.*m_pend.*cos(THE_Psi).*cos(THE_Theta).*cos(THE_Theta_pend).^2)./1.2e+1+(Ly_pend.^2.*m_pend.*cos(THE_Psi).*cos(THE_Theta).*cos(THE_Psi_pend).^2.*cos(THE_Theta_pend).^2)./1.2e+1-(Lz_pend.^2.*m_pend.*cos(THE_Psi).*cos(THE_Theta).*cos(THE_Psi_pend).^2.*cos(THE_Theta_pend).^2)./3.0-(Lx_pend.^2.*m_pend.*cos(THE_Phi_pend).*cos(THE_Theta_pend).*sin(THE_Theta).*sin(THE_Theta_pend))./1.2e+1+(Ly_pend.^2.*m_pend.*cos(THE_Phi_pend).*cos(THE_Theta_pend).*sin(THE_Theta).*sin(THE_Theta_pend))./1.2e+1+(Lz_pend.*Tv_Z_pend.*m_pend.*sin(THE_Theta).*sin(THE_Phi_pend).*sin(THE_Psi_pend))./2.0+(Lx_pend.^2.*m_pend.*cos(THE_Theta).*cos(THE_Theta_pend).*sin(THE_Psi).*sin(THE_Phi_pend).*sin(THE_Theta_pend))./1.2e+1-(Ly_pend.^2.*m_pend.*cos(THE_Theta).*cos(THE_Theta_pend).*sin(THE_Psi).*sin(THE_Phi_pend).*sin(THE_Theta_pend))./1.2e+1-(Ly_pend.^2.*m_pend.*cos(THE_Psi_pend).*cos(THE_Theta_pend).*sin(THE_Theta).*sin(THE_Phi_pend).*sin(THE_Psi_pend))./1.2e+1+(Lz_pend.^2.*m_pend.*cos(THE_Psi_pend).*cos(THE_Theta_pend).*sin(THE_Theta).*sin(THE_Phi_pend).*sin(THE_Psi_pend))./3.0+(Lz_pend.*Tv_Z_pend.*m_pend.*cos(THE_Theta).*cos(THE_Phi_pend).*sin(THE_Psi).*sin(THE_Psi_pend))./2.0+(Lz_pend.*Tv_Z_pend.*m_pend.*cos(THE_Phi_pend).*cos(THE_Psi_pend).*sin(THE_Theta).*sin(THE_Theta_pend))./2.0-(Ly_pend.^2.*m_pend.*cos(THE_Phi_pend).*cos(THE_Psi_pend).^2.*cos(THE_Theta_pend).*sin(THE_Theta).*sin(THE_Theta_pend))./1.2e+1+(Lz_pend.^2.*m_pend.*cos(THE_Phi_pend).*cos(THE_Psi_pend).^2.*cos(THE_Theta_pend).*sin(THE_Theta).*sin(THE_Theta_pend))./3.0-(Lz_pend.*Tv_Z_pend.*m_pend.*cos(THE_Theta).*cos(THE_Psi_pend).*sin(THE_Psi).*sin(THE_Phi_pend).*sin(THE_Theta_pend))./2.0+(Ly_pend.^2.*m_pend.*cos(THE_Theta).*cos(THE_Psi_pend).^2.*cos(THE_Theta_pend).*sin(THE_Psi).*sin(THE_Phi_pend).*sin(THE_Theta_pend))./1.2e+1-(Lz_pend.^2.*m_pend.*cos(THE_Theta).*cos(THE_Psi_pend).^2.*cos(THE_Theta_pend).*sin(THE_Psi).*sin(THE_Phi_pend).*sin(THE_Theta_pend))./3.0-(Ly_pend.^2.*m_pend.*cos(THE_Theta).*cos(THE_Phi_pend).*cos(THE_Psi_pend).*cos(THE_Theta_pend).*sin(THE_Psi).*sin(THE_Psi_pend))./1.2e+1+(Lz_pend.^2.*m_pend.*cos(THE_Theta).*cos(THE_Phi_pend).*cos(THE_Psi_pend).*cos(THE_Theta_pend).*sin(THE_Psi).*sin(THE_Psi_pend))./3.0,(Lx_pend.^2.*m_pend.*sin(THE_Theta).*sin(THE_Phi_pend))./1.2e+1+(Ly_pend.^2.*m_pend.*sin(THE_Theta).*sin(THE_Phi_pend))./1.2e+1-(Ly_pend.^2.*m_pend.*cos(THE_Psi_pend).^2.*sin(THE_Theta).*sin(THE_Phi_pend))./1.2e+1+(Lz_pend.^2.*m_pend.*cos(THE_Psi_pend).^2.*sin(THE_Theta).*sin(THE_Phi_pend))./3.0+(Lx_pend.^2.*m_pend.*cos(THE_Theta).*cos(THE_Phi_pend).*sin(THE_Psi))./1.2e+1+(Ly_pend.^2.*m_pend.*cos(THE_Theta).*cos(THE_Phi_pend).*sin(THE_Psi))./1.2e+1-(Ly_pend.^2.*m_pend.*cos(THE_Theta).*cos(THE_Phi_pend).*cos(THE_Psi_pend).^2.*sin(THE_Psi))./1.2e+1+(Lz_pend.^2.*m_pend.*cos(THE_Theta).*cos(THE_Phi_pend).*cos(THE_Psi_pend).^2.*sin(THE_Psi))./3.0-(Ly_pend.^2.*m_pend.*cos(THE_Psi).*cos(THE_Theta).*cos(THE_Psi_pend).*cos(THE_Theta_pend).*sin(THE_Psi_pend))./1.2e+1+(Lz_pend.^2.*m_pend.*cos(THE_Psi).*cos(THE_Theta).*cos(THE_Psi_pend).*cos(THE_Theta_pend).*sin(THE_Psi_pend))./3.0+(Ly_pend.^2.*m_pend.*cos(THE_Phi_pend).*cos(THE_Psi_pend).*sin(THE_Theta).*sin(THE_Psi_pend).*sin(THE_Theta_pend))./1.2e+1-(Lz_pend.^2.*m_pend.*cos(THE_Phi_pend).*cos(THE_Psi_pend).*sin(THE_Theta).*sin(THE_Psi_pend).*sin(THE_Theta_pend))./3.0+(Lz_pend.*Tv_Z_pend.*m_pend.*cos(THE_Psi_pend).*cos(THE_Theta_pend).*sin(THE_Theta).*sin(THE_Phi_pend))./2.0-(Ly_pend.^2.*m_pend.*cos(THE_Theta).*cos(THE_Psi_pend).*sin(THE_Psi).*sin(THE_Phi_pend).*sin(THE_Psi_pend).*sin(THE_Theta_pend))./1.2e+1+(Lz_pend.^2.*m_pend.*cos(THE_Theta).*cos(THE_Psi_pend).*sin(THE_Psi).*sin(THE_Phi_pend).*sin(THE_Psi_pend).*sin(THE_Theta_pend))./3.0+(Lz_pend.*Tv_Z_pend.*m_pend.*cos(THE_Theta).*cos(THE_Phi_pend).*cos(THE_Psi_pend).*cos(THE_Theta_pend).*sin(THE_Psi))./2.0,Ly_pend.^2.*m_pend.*cos(THE_Psi).*cos(THE_Theta).*sin(THE_Theta_pend).*(-1.0./1.2e+1)-(Ly_pend.^2.*m_pend.*cos(THE_Phi_pend).*cos(THE_Theta_pend).*sin(THE_Theta))./1.2e+1-(Lz_pend.^2.*m_pend.*cos(THE_Psi).*cos(THE_Theta).*sin(THE_Theta_pend))./3.0-(Lz_pend.^2.*m_pend.*cos(THE_Phi_pend).*cos(THE_Theta_pend).*sin(THE_Theta))./3.0+(Ly_pend.^2.*m_pend.*cos(THE_Theta).*cos(THE_Theta_pend).*sin(THE_Psi).*sin(THE_Phi_pend))./1.2e+1+(Lz_pend.^2.*m_pend.*cos(THE_Theta).*cos(THE_Theta_pend).*sin(THE_Psi).*sin(THE_Phi_pend))./3.0-(Lz_pend.*Tv_Z_pend.*m_pend.*cos(THE_Phi_pend).*cos(THE_Psi_pend).*sin(THE_Theta))./2.0+(Lz_pend.*Tv_Z_pend.*m_pend.*cos(THE_Theta).*cos(THE_Psi_pend).*sin(THE_Psi).*sin(THE_Phi_pend))./2.0-(Lz_pend.*Tv_Z_pend.*m_pend.*sin(THE_Theta).*sin(THE_Phi_pend).*sin(THE_Psi_pend).*sin(THE_Theta_pend))./2.0-(Lz_pend.*Tv_Z_pend.*m_pend.*cos(THE_Theta).*cos(THE_Phi_pend).*sin(THE_Psi).*sin(THE_Psi_pend).*sin(THE_Theta_pend))./2.0,-I_yz.*cos(THE_Theta)-Iprop_yz.*cos(THE_Theta).*4.0-I_xy.*cos(THE_Psi).*sin(THE_Theta)-Iprop_xy.*cos(THE_Psi).*sin(THE_Theta).*4.0+I_xz.*sin(THE_Psi).*sin(THE_Theta)+Iprop_xz.*sin(THE_Psi).*sin(THE_Theta).*4.0+I_yz.*cos(THE_Psi).^2.*cos(THE_Theta).*2.0+Iprop_yz.*cos(THE_Psi).^2.*cos(THE_Theta).*8.0+I_yy.*cos(THE_Psi).*cos(THE_Theta).*sin(THE_Psi)-I_zz.*cos(THE_Psi).*cos(THE_Theta).*sin(THE_Psi)+Iprop_yy.*cos(THE_Psi).*cos(THE_Theta).*sin(THE_Psi).*4.0-Iprop_zz.*cos(THE_Psi).*cos(THE_Theta).*sin(THE_Psi).*4.0+(Lx_pend.^2.*m_pend.*cos(THE_Psi).*cos(THE_Theta).*sin(THE_Psi))./1.2e+1-(Ly_pend.^2.*m_pend.*cos(THE_Psi).*cos(THE_Theta).*sin(THE_Psi))./1.2e+1+Tv_Z_pend.^2.*m_pend.*cos(THE_Psi).*cos(THE_Theta).*sin(THE_Psi)+cg_to_mot_H.^2.*mprop.*cos(THE_Psi).*cos(THE_Theta).*sin(THE_Psi).*4.0-cg_to_mot_L.^2.*mprop.*cos(THE_Psi).*cos(THE_Theta).*sin(THE_Psi).*2.0-(Lx_pend.^2.*m_pend.*cos(THE_Theta).*cos(THE_Theta_pend).*sin(THE_Phi_pend).*sin(THE_Theta_pend))./1.2e+1+(Ly_pend.^2.*m_pend.*cos(THE_Psi).*cos(THE_Phi_pend).*sin(THE_Theta).*sin(THE_Phi_pend))./1.2e+1+(Ly_pend.^2.*m_pend.*cos(THE_Theta).*cos(THE_Theta_pend).*sin(THE_Phi_pend).*sin(THE_Theta_pend))./1.2e+1-(Lz_pend.^2.*m_pend.*cos(THE_Psi).*cos(THE_Phi_pend).*sin(THE_Theta).*sin(THE_Phi_pend))./3.0-(Lz_pend.*Tv_Z_pend.*m_pend.*cos(THE_Theta).*cos(THE_Phi_pend).*sin(THE_Psi_pend))./2.0-(Lx_pend.^2.*m_pend.*cos(THE_Psi).*cos(THE_Theta).*cos(THE_Theta_pend).^2.*sin(THE_Psi))./6.0+(Ly_pend.^2.*m_pend.*cos(THE_Psi).*cos(THE_Theta).*cos(THE_Phi_pend).^2.*sin(THE_Psi))./1.2e+1+(Ly_pend.^2.*m_pend.*cos(THE_Psi).*cos(THE_Theta).*cos(THE_Psi_pend).^2.*sin(THE_Psi))./1.2e+1+(Ly_pend.^2.*m_pend.*cos(THE_Psi).*cos(THE_Theta).*cos(THE_Theta_pend).^2.*sin(THE_Psi))./6.0-(Lz_pend.^2.*m_pend.*cos(THE_Psi).*cos(THE_Theta).*cos(THE_Phi_pend).^2.*sin(THE_Psi))./3.0-(Lz_pend.^2.*m_pend.*cos(THE_Psi).*cos(THE_Theta).*cos(THE_Psi_pend).^2.*sin(THE_Psi))./3.0+(Ly_pend.^2.*m_pend.*cos(THE_Theta).*cos(THE_Phi_pend).*cos(THE_Psi_pend).*cos(THE_Theta_pend).*sin(THE_Psi_pend))./1.2e+1-(Lz_pend.^2.*m_pend.*cos(THE_Theta).*cos(THE_Phi_pend).*cos(THE_Psi_pend).*cos(THE_Theta_pend).*sin(THE_Psi_pend))./3.0+(Lx_pend.^2.*m_pend.*cos(THE_Phi_pend).*cos(THE_Theta_pend).*sin(THE_Psi).*sin(THE_Theta).*sin(THE_Theta_pend))./1.2e+1-(Ly_pend.^2.*m_pend.*cos(THE_Psi).*cos(THE_Psi_pend).*sin(THE_Theta).*sin(THE_Psi_pend).*sin(THE_Theta_pend))./1.2e+1-(Ly_pend.^2.*m_pend.*cos(THE_Phi_pend).*cos(THE_Theta_pend).*sin(THE_Psi).*sin(THE_Theta).*sin(THE_Theta_pend))./1.2e+1+(Lz_pend.^2.*m_pend.*cos(THE_Psi).*cos(THE_Psi_pend).*sin(THE_Theta).*sin(THE_Psi_pend).*sin(THE_Theta_pend))./3.0+(Lz_pend.*Tv_Z_pend.*m_pend.*cos(THE_Theta).*cos(THE_Psi_pend).*sin(THE_Phi_pend).*sin(THE_Theta_pend))./2.0-(Lz_pend.*Tv_Z_pend.*m_pend.*sin(THE_Psi).*sin(THE_Theta).*sin(THE_Phi_pend).*sin(THE_Psi_pend))./2.0+(Lx_pend.^2.*m_pend.*cos(THE_Psi).*cos(THE_Phi_pend).*cos(THE_Theta_pend).^2.*sin(THE_Theta).*sin(THE_Phi_pend))./1.2e+1+(Lx_pend.^2.*m_pend.*cos(THE_Psi).^2.*cos(THE_Theta).*cos(THE_Theta_pend).*sin(THE_Phi_pend).*sin(THE_Theta_pend))./6.0-(Ly_pend.^2.*m_pend.*cos(THE_Psi).*cos(THE_Phi_pend).*cos(THE_Psi_pend).^2.*sin(THE_Theta).*sin(THE_Phi_pend))./6.0-(Ly_pend.^2.*m_pend.*cos(THE_Psi).*cos(THE_Phi_pend).*cos(THE_Theta_pend).^2.*sin(THE_Theta).*sin(THE_Phi_pend))./1.2e+1-(Ly_pend.^2.*m_pend.*cos(THE_Psi).^2.*cos(THE_Theta).*cos(THE_Theta_pend).*sin(THE_Phi_pend).*sin(THE_Theta_pend))./6.0-(Ly_pend.^2.*m_pend.*cos(THE_Theta).*cos(THE_Psi_pend).^2.*cos(THE_Theta_pend).*sin(THE_Phi_pend).*sin(THE_Theta_pend))./1.2e+1+Lz_pend.^2.*m_pend.*cos(THE_Psi).*cos(THE_Phi_pend).*cos(THE_Psi_pend).^2.*sin(THE_Theta).*sin(THE_Phi_pend).*(2.0./3.0)+(Lz_pend.^2.*m_pend.*cos(THE_Theta).*cos(THE_Psi_pend).^2.*cos(THE_Theta_pend).*sin(THE_Phi_pend).*sin(THE_Theta_pend))./3.0+Lz_pend.*Tv_Z_pend.*m_pend.*cos(THE_Psi).^2.*cos(THE_Theta).*cos(THE_Phi_pend).*sin(THE_Psi_pend)+(Lx_pend.^2.*m_pend.*cos(THE_Psi).*cos(THE_Theta).*cos(THE_Phi_pend).^2.*cos(THE_Theta_pend).^2.*sin(THE_Psi))./1.2e+1-(Ly_pend.^2.*m_pend.*cos(THE_Psi).*cos(THE_Theta).*cos(THE_Phi_pend).^2.*cos(THE_Psi_pend).^2.*sin(THE_Psi))./6.0-(Ly_pend.^2.*m_pend.*cos(THE_Psi).*cos(THE_Theta).*cos(THE_Phi_pend).^2.*cos(THE_Theta_pend).^2.*sin(THE_Psi))./1.2e+1-(Ly_pend.^2.*m_pend.*cos(THE_Psi).*cos(THE_Theta).*cos(THE_Psi_pend).^2.*cos(THE_Theta_pend).^2.*sin(THE_Psi))./6.0+Lz_pend.^2.*m_pend.*cos(THE_Psi).*cos(THE_Theta).*cos(THE_Phi_pend).^2.*cos(THE_Psi_pend).^2.*sin(THE_Psi).*(2.0./3.0)+Lz_pend.^2.*m_pend.*cos(THE_Psi).*cos(THE_Theta).*cos(THE_Psi_pend).^2.*cos(THE_Theta_pend).^2.*sin(THE_Psi).*(2.0./3.0)+(Ly_pend.^2.*m_pend.*cos(THE_Psi_pend).*cos(THE_Theta_pend).*sin(THE_Psi).*sin(THE_Theta).*sin(THE_Phi_pend).*sin(THE_Psi_pend))./1.2e+1-(Lz_pend.^2.*m_pend.*cos(THE_Psi_pend).*cos(THE_Theta_pend).*sin(THE_Psi).*sin(THE_Theta).*sin(THE_Phi_pend).*sin(THE_Psi_pend))./3.0+Lz_pend.*Tv_Z_pend.*m_pend.*cos(THE_Psi).*cos(THE_Theta).*cos(THE_Psi_pend).*cos(THE_Theta_pend).*sin(THE_Psi)-(Lz_pend.*Tv_Z_pend.*m_pend.*cos(THE_Phi_pend).*cos(THE_Psi_pend).*sin(THE_Psi).*sin(THE_Theta).*sin(THE_Theta_pend))./2.0-(Ly_pend.^2.*m_pend.*cos(THE_Psi).^2.*cos(THE_Theta).*cos(THE_Phi_pend).*cos(THE_Psi_pend).*cos(THE_Theta_pend).*sin(THE_Psi_pend))./6.0+Lz_pend.^2.*m_pend.*cos(THE_Psi).^2.*cos(THE_Theta).*cos(THE_Phi_pend).*cos(THE_Psi_pend).*cos(THE_Theta_pend).*sin(THE_Psi_pend).*(2.0./3.0)+(Ly_pend.^2.*m_pend.*cos(THE_Psi).*cos(THE_Phi_pend).^2.*cos(THE_Psi_pend).*sin(THE_Theta).*sin(THE_Psi_pend).*sin(THE_Theta_pend))./6.0+(Ly_pend.^2.*m_pend.*cos(THE_Phi_pend).*cos(THE_Psi_pend).^2.*cos(THE_Theta_pend).*sin(THE_Psi).*sin(THE_Theta).*sin(THE_Theta_pend))./1.2e+1-Lz_pend.^2.*m_pend.*cos(THE_Psi).*cos(THE_Phi_pend).^2.*cos(THE_Psi_pend).*sin(THE_Theta).*sin(THE_Psi_pend).*sin(THE_Theta_pend).*(2.0./3.0)-(Lz_pend.^2.*m_pend.*cos(THE_Phi_pend).*cos(THE_Psi_pend).^2.*cos(THE_Theta_pend).*sin(THE_Psi).*sin(THE_Theta).*sin(THE_Theta_pend))./3.0-Lz_pend.*Tv_Z_pend.*m_pend.*cos(THE_Psi).^2.*cos(THE_Theta).*cos(THE_Psi_pend).*sin(THE_Phi_pend).*sin(THE_Theta_pend)+(Ly_pend.^2.*m_pend.*cos(THE_Psi).*cos(THE_Phi_pend).*cos(THE_Psi_pend).^2.*cos(THE_Theta_pend).^2.*sin(THE_Theta).*sin(THE_Phi_pend))./1.2e+1+(Ly_pend.^2.*m_pend.*cos(THE_Psi).^2.*cos(THE_Theta).*cos(THE_Psi_pend).^2.*cos(THE_Theta_pend).*sin(THE_Phi_pend).*sin(THE_Theta_pend))./6.0-(Lz_pend.^2.*m_pend.*cos(THE_Psi).*cos(THE_Phi_pend).*cos(THE_Psi_pend).^2.*cos(THE_Theta_pend).^2.*sin(THE_Theta).*sin(THE_Phi_pend))./3.0-Lz_pend.^2.*m_pend.*cos(THE_Psi).^2.*cos(THE_Theta).*cos(THE_Psi_pend).^2.*cos(THE_Theta_pend).*sin(THE_Phi_pend).*sin(THE_Theta_pend).*(2.0./3.0)+(Ly_pend.^2.*m_pend.*cos(THE_Psi).*cos(THE_Theta).*cos(THE_Phi_pend).^2.*cos(THE_Psi_pend).^2.*cos(THE_Theta_pend).^2.*sin(THE_Psi))./1.2e+1-(Lz_pend.^2.*m_pend.*cos(THE_Psi).*cos(THE_Theta).*cos(THE_Phi_pend).^2.*cos(THE_Psi_pend).^2.*cos(THE_Theta_pend).^2.*sin(THE_Psi))./3.0-(Ly_pend.^2.*m_pend.*cos(THE_Psi).*cos(THE_Theta).*cos(THE_Phi_pend).*cos(THE_Psi_pend).*sin(THE_Psi).*sin(THE_Phi_pend).*sin(THE_Psi_pend).*sin(THE_Theta_pend))./6.0+Lz_pend.^2.*m_pend.*cos(THE_Psi).*cos(THE_Theta).*cos(THE_Phi_pend).*cos(THE_Psi_pend).*sin(THE_Psi).*sin(THE_Phi_pend).*sin(THE_Psi_pend).*sin(THE_Theta_pend).*(2.0./3.0),I_zz+Iprop_zz.*4.0+(Ly_pend.^2.*m_pend)./1.2e+1+(Lz_pend.^2.*m_pend)./3.0+cg_to_mot_L.^2.*mprop.*4.0+I_yy.*cos(THE_Psi).^2-I_zz.*cos(THE_Psi).^2+Iprop_yy.*cos(THE_Psi).^2.*4.0-Iprop_zz.*cos(THE_Psi).^2.*4.0-I_yz.*sin(THE_Psi.*2.0)-Iprop_yz.*sin(THE_Psi.*2.0).*4.0+(Lx_pend.^2.*m_pend.*cos(THE_Psi).^2)./1.2e+1+(Lx_pend.^2.*m_pend.*cos(THE_Theta_pend).^2)./1.2e+1-(Ly_pend.^2.*m_pend.*cos(THE_Psi).^2)./1.2e+1-(Ly_pend.^2.*m_pend.*cos(THE_Theta_pend).^2)./1.2e+1+Tv_Z_pend.^2.*m_pend.*cos(THE_Psi).^2+cg_to_mot_H.^2.*mprop.*cos(THE_Psi).^2.*4.0-cg_to_mot_L.^2.*mprop.*cos(THE_Psi).^2.*2.0-(Lx_pend.^2.*m_pend.*cos(THE_Psi).^2.*cos(THE_Theta_pend).^2)./6.0+(Ly_pend.^2.*m_pend.*cos(THE_Psi).^2.*cos(THE_Phi_pend).^2)./1.2e+1+(Ly_pend.^2.*m_pend.*cos(THE_Psi).^2.*cos(THE_Psi_pend).^2)./1.2e+1+(Ly_pend.^2.*m_pend.*cos(THE_Psi).^2.*cos(THE_Theta_pend).^2)./6.0+(Ly_pend.^2.*m_pend.*cos(THE_Psi_pend).^2.*cos(THE_Theta_pend).^2)./1.2e+1-(Lz_pend.^2.*m_pend.*cos(THE_Psi).^2.*cos(THE_Phi_pend).^2)./3.0-(Lz_pend.^2.*m_pend.*cos(THE_Psi).^2.*cos(THE_Psi_pend).^2)./3.0-(Lz_pend.^2.*m_pend.*cos(THE_Psi_pend).^2.*cos(THE_Theta_pend).^2)./3.0+(Lx_pend.^2.*m_pend.*cos(THE_Psi).^2.*cos(THE_Phi_pend).^2.*cos(THE_Theta_pend).^2)./1.2e+1-(Ly_pend.^2.*m_pend.*cos(THE_Psi).^2.*cos(THE_Phi_pend).^2.*cos(THE_Psi_pend).^2)./6.0-(Ly_pend.^2.*m_pend.*cos(THE_Psi).^2.*cos(THE_Phi_pend).^2.*cos(THE_Theta_pend).^2)./1.2e+1-(Ly_pend.^2.*m_pend.*cos(THE_Psi).^2.*cos(THE_Psi_pend).^2.*cos(THE_Theta_pend).^2)./6.0+Lz_pend.^2.*m_pend.*cos(THE_Psi).^2.*cos(THE_Phi_pend).^2.*cos(THE_Psi_pend).^2.*(2.0./3.0)+Lz_pend.^2.*m_pend.*cos(THE_Psi).^2.*cos(THE_Psi_pend).^2.*cos(THE_Theta_pend).^2.*(2.0./3.0)+(Ly_pend.^2.*m_pend.*cos(THE_Psi).^2.*cos(THE_Phi_pend).^2.*cos(THE_Psi_pend).^2.*cos(THE_Theta_pend).^2)./1.2e+1-(Lz_pend.^2.*m_pend.*cos(THE_Psi).^2.*cos(THE_Phi_pend).^2.*cos(THE_Psi_pend).^2.*cos(THE_Theta_pend).^2)./3.0+Lz_pend.*Tv_Z_pend.*m_pend.*cos(THE_Psi).^2.*cos(THE_Psi_pend).*cos(THE_Theta_pend)-(Lx_pend.^2.*m_pend.*cos(THE_Psi).*cos(THE_Theta_pend).*sin(THE_Psi).*sin(THE_Phi_pend).*sin(THE_Theta_pend))./6.0+(Ly_pend.^2.*m_pend.*cos(THE_Psi).*cos(THE_Theta_pend).*sin(THE_Psi).*sin(THE_Phi_pend).*sin(THE_Theta_pend))./6.0-Lz_pend.*Tv_Z_pend.*m_pend.*cos(THE_Psi).*cos(THE_Phi_pend).*sin(THE_Psi).*sin(THE_Psi_pend)+Lz_pend.*Tv_Z_pend.*m_pend.*cos(THE_Psi).*cos(THE_Psi_pend).*sin(THE_Psi).*sin(THE_Phi_pend).*sin(THE_Theta_pend)-(Ly_pend.^2.*m_pend.*cos(THE_Psi).*cos(THE_Psi_pend).^2.*cos(THE_Theta_pend).*sin(THE_Psi).*sin(THE_Phi_pend).*sin(THE_Theta_pend))./6.0-(Ly_pend.^2.*m_pend.*cos(THE_Psi).^2.*cos(THE_Phi_pend).*cos(THE_Psi_pend).*sin(THE_Phi_pend).*sin(THE_Psi_pend).*sin(THE_Theta_pend))./6.0+Lz_pend.^2.*m_pend.*cos(THE_Psi).*cos(THE_Psi_pend).^2.*cos(THE_Theta_pend).*sin(THE_Psi).*sin(THE_Phi_pend).*sin(THE_Theta_pend).*(2.0./3.0)+Lz_pend.^2.*m_pend.*cos(THE_Psi).^2.*cos(THE_Phi_pend).*cos(THE_Psi_pend).*sin(THE_Phi_pend).*sin(THE_Psi_pend).*sin(THE_Theta_pend).*(2.0./3.0)+(Ly_pend.^2.*m_pend.*cos(THE_Psi).*cos(THE_Phi_pend).*cos(THE_Psi_pend).*cos(THE_Theta_pend).*sin(THE_Psi).*sin(THE_Psi_pend))./6.0-Lz_pend.^2.*m_pend.*cos(THE_Psi).*cos(THE_Phi_pend).*cos(THE_Psi_pend).*cos(THE_Theta_pend).*sin(THE_Psi).*sin(THE_Psi_pend).*(2.0./3.0),I_xy.*cos(THE_Psi)+Iprop_xy.*cos(THE_Psi).*4.0-I_xz.*sin(THE_Psi)-Iprop_xz.*sin(THE_Psi).*4.0-(Ly_pend.^2.*m_pend.*cos(THE_Psi).*cos(THE_Phi_pend).*sin(THE_Phi_pend))./1.2e+1+(Lz_pend.^2.*m_pend.*cos(THE_Psi).*cos(THE_Phi_pend).*sin(THE_Phi_pend))./3.0-(Lx_pend.^2.*m_pend.*cos(THE_Phi_pend).*cos(THE_Theta_pend).*sin(THE_Psi).*sin(THE_Theta_pend))./1.2e+1+(Ly_pend.^2.*m_pend.*cos(THE_Psi).*cos(THE_Psi_pend).*sin(THE_Psi_pend).*sin(THE_Theta_pend))./1.2e+1+(Ly_pend.^2.*m_pend.*cos(THE_Phi_pend).*cos(THE_Theta_pend).*sin(THE_Psi).*sin(THE_Theta_pend))./1.2e+1-(Lz_pend.^2.*m_pend.*cos(THE_Psi).*cos(THE_Psi_pend).*sin(THE_Psi_pend).*sin(THE_Theta_pend))./3.0+(Lz_pend.*Tv_Z_pend.*m_pend.*sin(THE_Psi).*sin(THE_Phi_pend).*sin(THE_Psi_pend))./2.0-(Lx_pend.^2.*m_pend.*cos(THE_Psi).*cos(THE_Phi_pend).*cos(THE_Theta_pend).^2.*sin(THE_Phi_pend))./1.2e+1+(Ly_pend.^2.*m_pend.*cos(THE_Psi).*cos(THE_Phi_pend).*cos(THE_Psi_pend).^2.*sin(THE_Phi_pend))./6.0+(Ly_pend.^2.*m_pend.*cos(THE_Psi).*cos(THE_Phi_pend).*cos(THE_Theta_pend).^2.*sin(THE_Phi_pend))./1.2e+1-Lz_pend.^2.*m_pend.*cos(THE_Psi).*cos(THE_Phi_pend).*cos(THE_Psi_pend).^2.*sin(THE_Phi_pend).*(2.0./3.0)-(Ly_pend.^2.*m_pend.*cos(THE_Psi_pend).*cos(THE_Theta_pend).*sin(THE_Psi).*sin(THE_Phi_pend).*sin(THE_Psi_pend))./1.2e+1+(Lz_pend.^2.*m_pend.*cos(THE_Psi_pend).*cos(THE_Theta_pend).*sin(THE_Psi).*sin(THE_Phi_pend).*sin(THE_Psi_pend))./3.0+(Lz_pend.*Tv_Z_pend.*m_pend.*cos(THE_Phi_pend).*cos(THE_Psi_pend).*sin(THE_Psi).*sin(THE_Theta_pend))./2.0-(Ly_pend.^2.*m_pend.*cos(THE_Psi).*cos(THE_Phi_pend).^2.*cos(THE_Psi_pend).*sin(THE_Psi_pend).*sin(THE_Theta_pend))./6.0-(Ly_pend.^2.*m_pend.*cos(THE_Phi_pend).*cos(THE_Psi_pend).^2.*cos(THE_Theta_pend).*sin(THE_Psi).*sin(THE_Theta_pend))./1.2e+1+Lz_pend.^2.*m_pend.*cos(THE_Psi).*cos(THE_Phi_pend).^2.*cos(THE_Psi_pend).*sin(THE_Psi_pend).*sin(THE_Theta_pend).*(2.0./3.0)+(Lz_pend.^2.*m_pend.*cos(THE_Phi_pend).*cos(THE_Psi_pend).^2.*cos(THE_Theta_pend).*sin(THE_Psi).*sin(THE_Theta_pend))./3.0-(Ly_pend.^2.*m_pend.*cos(THE_Psi).*cos(THE_Phi_pend).*cos(THE_Psi_pend).^2.*cos(THE_Theta_pend).^2.*sin(THE_Phi_pend))./1.2e+1+(Lz_pend.^2.*m_pend.*cos(THE_Psi).*cos(THE_Phi_pend).*cos(THE_Psi_pend).^2.*cos(THE_Theta_pend).^2.*sin(THE_Phi_pend))./3.0,(cos(THE_Phi).*(Tv_Z_pend.*m_pend.*cos(THE_Psi).*cos(THE_Theta).*2.0+cg_to_mot_H.*mprop.*cos(THE_Psi).*cos(THE_Theta).*8.0-Lz_pend.*m_pend.*sin(THE_Theta).*sin(THE_Phi_pend).*sin(THE_Psi_pend)-Lz_pend.*m_pend.*cos(THE_Theta).*cos(THE_Phi_pend).*sin(THE_Psi).*sin(THE_Psi_pend)-Lz_pend.*m_pend.*cos(THE_Phi_pend).*cos(THE_Psi_pend).*sin(THE_Theta).*sin(THE_Theta_pend)+Lz_pend.*m_pend.*cos(THE_Psi).*cos(THE_Theta).*cos(THE_Psi_pend).*cos(THE_Theta_pend)+Lz_pend.*m_pend.*cos(THE_Theta).*cos(THE_Psi_pend).*sin(THE_Psi).*sin(THE_Phi_pend).*sin(THE_Theta_pend)))./2.0,(sin(THE_Phi).*(Tv_Z_pend.*m_pend.*cos(THE_Psi).*cos(THE_Theta).*2.0+cg_to_mot_H.*mprop.*cos(THE_Psi).*cos(THE_Theta).*8.0-Lz_pend.*m_pend.*sin(THE_Theta).*sin(THE_Phi_pend).*sin(THE_Psi_pend)-Lz_pend.*m_pend.*cos(THE_Theta).*cos(THE_Phi_pend).*sin(THE_Psi).*sin(THE_Psi_pend)-Lz_pend.*m_pend.*cos(THE_Phi_pend).*cos(THE_Psi_pend).*sin(THE_Theta).*sin(THE_Theta_pend)+Lz_pend.*m_pend.*cos(THE_Psi).*cos(THE_Theta).*cos(THE_Psi_pend).*cos(THE_Theta_pend)+Lz_pend.*m_pend.*cos(THE_Theta).*cos(THE_Psi_pend).*sin(THE_Psi).*sin(THE_Phi_pend).*sin(THE_Theta_pend)))./2.0,-Tv_Z_pend.*m_pend.*cos(THE_Psi).*sin(THE_Theta)-cg_to_mot_H.*mprop.*cos(THE_Psi).*sin(THE_Theta).*4.0-(Lz_pend.*m_pend.*cos(THE_Theta).*sin(THE_Phi_pend).*sin(THE_Psi_pend))./2.0-(Lz_pend.*m_pend.*cos(THE_Psi).*cos(THE_Psi_pend).*cos(THE_Theta_pend).*sin(THE_Theta))./2.0-(Lz_pend.*m_pend.*cos(THE_Theta).*cos(THE_Phi_pend).*cos(THE_Psi_pend).*sin(THE_Theta_pend))./2.0+(Lz_pend.*m_pend.*cos(THE_Phi_pend).*sin(THE_Psi).*sin(THE_Theta).*sin(THE_Psi_pend))./2.0-(Lz_pend.*m_pend.*cos(THE_Psi_pend).*sin(THE_Psi).*sin(THE_Theta).*sin(THE_Phi_pend).*sin(THE_Theta_pend))./2.0,Ly_pend.^2.*m_pend.*sin(THE_Psi).*(-1.0./1.2e+1)-(Lz_pend.^2.*m_pend.*sin(THE_Psi))./3.0-(Lx_pend.^2.*m_pend.*cos(THE_Theta_pend).^2.*sin(THE_Psi))./1.2e+1+(Ly_pend.^2.*m_pend.*cos(THE_Theta_pend).^2.*sin(THE_Psi))./1.2e+1-(Ly_pend.^2.*m_pend.*cos(THE_Psi_pend).^2.*cos(THE_Theta_pend).^2.*sin(THE_Psi))./1.2e+1+(Lz_pend.^2.*m_pend.*cos(THE_Psi_pend).^2.*cos(THE_Theta_pend).^2.*sin(THE_Psi))./3.0+(Lx_pend.^2.*m_pend.*cos(THE_Psi).*cos(THE_Theta_pend).*sin(THE_Phi_pend).*sin(THE_Theta_pend))./1.2e+1-(Ly_pend.^2.*m_pend.*cos(THE_Psi).*cos(THE_Theta_pend).*sin(THE_Phi_pend).*sin(THE_Theta_pend))./1.2e+1+(Lz_pend.*Tv_Z_pend.*m_pend.*cos(THE_Psi).*cos(THE_Phi_pend).*sin(THE_Psi_pend))./2.0-(Ly_pend.^2.*m_pend.*cos(THE_Psi).*cos(THE_Phi_pend).*cos(THE_Psi_pend).*cos(THE_Theta_pend).*sin(THE_Psi_pend))./1.2e+1+(Lz_pend.^2.*m_pend.*cos(THE_Psi).*cos(THE_Phi_pend).*cos(THE_Psi_pend).*cos(THE_Theta_pend).*sin(THE_Psi_pend))./3.0-(Lz_pend.*Tv_Z_pend.*m_pend.*cos(THE_Psi).*cos(THE_Psi_pend).*sin(THE_Phi_pend).*sin(THE_Theta_pend))./2.0+(Ly_pend.^2.*m_pend.*cos(THE_Psi).*cos(THE_Psi_pend).^2.*cos(THE_Theta_pend).*sin(THE_Phi_pend).*sin(THE_Theta_pend))./1.2e+1-(Lz_pend.^2.*m_pend.*cos(THE_Psi).*cos(THE_Psi_pend).^2.*cos(THE_Theta_pend).*sin(THE_Phi_pend).*sin(THE_Theta_pend))./3.0,(Lx_pend.^2.*m_pend.*cos(THE_Psi).*cos(THE_Phi_pend))./1.2e+1+(Ly_pend.^2.*m_pend.*cos(THE_Psi).*cos(THE_Phi_pend))./1.2e+1-(Ly_pend.^2.*m_pend.*cos(THE_Psi).*cos(THE_Phi_pend).*cos(THE_Psi_pend).^2)./1.2e+1+(Lz_pend.^2.*m_pend.*cos(THE_Psi).*cos(THE_Phi_pend).*cos(THE_Psi_pend).^2)./3.0+(Ly_pend.^2.*m_pend.*cos(THE_Psi_pend).*cos(THE_Theta_pend).*sin(THE_Psi).*sin(THE_Psi_pend))./1.2e+1-(Lz_pend.^2.*m_pend.*cos(THE_Psi_pend).*cos(THE_Theta_pend).*sin(THE_Psi).*sin(THE_Psi_pend))./3.0-(Ly_pend.^2.*m_pend.*cos(THE_Psi).*cos(THE_Psi_pend).*sin(THE_Phi_pend).*sin(THE_Psi_pend).*sin(THE_Theta_pend))./1.2e+1+(Lz_pend.^2.*m_pend.*cos(THE_Psi).*cos(THE_Psi_pend).*sin(THE_Phi_pend).*sin(THE_Psi_pend).*sin(THE_Theta_pend))./3.0+(Lz_pend.*Tv_Z_pend.*m_pend.*cos(THE_Psi).*cos(THE_Phi_pend).*cos(THE_Psi_pend).*cos(THE_Theta_pend))./2.0,(Ly_pend.^2.*m_pend.*sin(THE_Psi).*sin(THE_Theta_pend))./1.2e+1+(Lz_pend.^2.*m_pend.*sin(THE_Psi).*sin(THE_Theta_pend))./3.0+(Ly_pend.^2.*m_pend.*cos(THE_Psi).*cos(THE_Theta_pend).*sin(THE_Phi_pend))./1.2e+1+(Lz_pend.^2.*m_pend.*cos(THE_Psi).*cos(THE_Theta_pend).*sin(THE_Phi_pend))./3.0+(Lz_pend.*Tv_Z_pend.*m_pend.*cos(THE_Psi).*cos(THE_Psi_pend).*sin(THE_Phi_pend))./2.0-(Lz_pend.*Tv_Z_pend.*m_pend.*cos(THE_Psi).*cos(THE_Phi_pend).*sin(THE_Psi_pend).*sin(THE_Theta_pend))./2.0,-I_xx.*sin(THE_Theta)-Iprop_xx.*sin(THE_Theta).*4.0+I_xz.*cos(THE_Psi).*cos(THE_Theta)+Iprop_xz.*cos(THE_Psi).*cos(THE_Theta).*4.0+I_xy.*cos(THE_Theta).*sin(THE_Psi)+Iprop_xy.*cos(THE_Theta).*sin(THE_Psi).*4.0-(Lx_pend.^2.*m_pend.*sin(THE_Theta))./1.2e+1-(Ly_pend.^2.*m_pend.*sin(THE_Theta))./1.2e+1-Tv_Z_pend.^2.*m_pend.*sin(THE_Theta)-cg_to_mot_H.^2.*mprop.*sin(THE_Theta).*4.0-cg_to_mot_L.^2.*mprop.*sin(THE_Theta).*2.0+(Ly_pend.^2.*m_pend.*cos(THE_Phi_pend).^2.*sin(THE_Theta))./1.2e+1+(Ly_pend.^2.*m_pend.*cos(THE_Psi_pend).^2.*sin(THE_Theta))./1.2e+1-(Lz_pend.^2.*m_pend.*cos(THE_Phi_pend).^2.*sin(THE_Theta))./3.0-(Lz_pend.^2.*m_pend.*cos(THE_Psi_pend).^2.*sin(THE_Theta))./3.0+(Lx_pend.^2.*m_pend.*cos(THE_Phi_pend).^2.*cos(THE_Theta_pend).^2.*sin(THE_Theta))./1.2e+1-(Ly_pend.^2.*m_pend.*cos(THE_Phi_pend).^2.*cos(THE_Psi_pend).^2.*sin(THE_Theta))./6.0-(Ly_pend.^2.*m_pend.*cos(THE_Phi_pend).^2.*cos(THE_Theta_pend).^2.*sin(THE_Theta))./1.2e+1+Lz_pend.^2.*m_pend.*cos(THE_Phi_pend).^2.*cos(THE_Psi_pend).^2.*sin(THE_Theta).*(2.0./3.0)-(Ly_pend.^2.*m_pend.*cos(THE_Theta).*cos(THE_Phi_pend).*sin(THE_Psi).*sin(THE_Phi_pend))./1.2e+1+(Lz_pend.^2.*m_pend.*cos(THE_Theta).*cos(THE_Phi_pend).*sin(THE_Psi).*sin(THE_Phi_pend))./3.0+(Ly_pend.^2.*m_pend.*cos(THE_Phi_pend).^2.*cos(THE_Psi_pend).^2.*cos(THE_Theta_pend).^2.*sin(THE_Theta))./1.2e+1-(Lz_pend.^2.*m_pend.*cos(THE_Phi_pend).^2.*cos(THE_Psi_pend).^2.*cos(THE_Theta_pend).^2.*sin(THE_Theta))./3.0-Lz_pend.*Tv_Z_pend.*m_pend.*cos(THE_Psi_pend).*cos(THE_Theta_pend).*sin(THE_Theta)+(Lx_pend.^2.*m_pend.*cos(THE_Psi).*cos(THE_Theta).*cos(THE_Phi_pend).*cos(THE_Theta_pend).*sin(THE_Theta_pend))./1.2e+1-(Ly_pend.^2.*m_pend.*cos(THE_Psi).*cos(THE_Theta).*cos(THE_Phi_pend).*cos(THE_Theta_pend).*sin(THE_Theta_pend))./1.2e+1+(Ly_pend.^2.*m_pend.*cos(THE_Theta).*cos(THE_Psi_pend).*sin(THE_Psi).*sin(THE_Psi_pend).*sin(THE_Theta_pend))./1.2e+1-(Lz_pend.^2.*m_pend.*cos(THE_Theta).*cos(THE_Psi_pend).*sin(THE_Psi).*sin(THE_Psi_pend).*sin(THE_Theta_pend))./3.0-(Lz_pend.*Tv_Z_pend.*m_pend.*cos(THE_Psi).*cos(THE_Theta).*sin(THE_Phi_pend).*sin(THE_Psi_pend))./2.0-(Lx_pend.^2.*m_pend.*cos(THE_Theta).*cos(THE_Phi_pend).*cos(THE_Theta_pend).^2.*sin(THE_Psi).*sin(THE_Phi_pend))./1.2e+1+(Ly_pend.^2.*m_pend.*cos(THE_Theta).*cos(THE_Phi_pend).*cos(THE_Psi_pend).^2.*sin(THE_Psi).*sin(THE_Phi_pend))./6.0+(Ly_pend.^2.*m_pend.*cos(THE_Theta).*cos(THE_Phi_pend).*cos(THE_Theta_pend).^2.*sin(THE_Psi).*sin(THE_Phi_pend))./1.2e+1-Lz_pend.^2.*m_pend.*cos(THE_Theta).*cos(THE_Phi_pend).*cos(THE_Psi_pend).^2.*sin(THE_Psi).*sin(THE_Phi_pend).*(2.0./3.0)-(Ly_pend.^2.*m_pend.*cos(THE_Phi_pend).*cos(THE_Psi_pend).*sin(THE_Theta).*sin(THE_Phi_pend).*sin(THE_Psi_pend).*sin(THE_Theta_pend))./6.0+Lz_pend.^2.*m_pend.*cos(THE_Phi_pend).*cos(THE_Psi_pend).*sin(THE_Theta).*sin(THE_Phi_pend).*sin(THE_Psi_pend).*sin(THE_Theta_pend).*(2.0./3.0)-(Lz_pend.*Tv_Z_pend.*m_pend.*cos(THE_Psi).*cos(THE_Theta).*cos(THE_Phi_pend).*cos(THE_Psi_pend).*sin(THE_Theta_pend))./2.0+(Ly_pend.^2.*m_pend.*cos(THE_Psi).*cos(THE_Theta).*cos(THE_Phi_pend).*cos(THE_Psi_pend).^2.*cos(THE_Theta_pend).*sin(THE_Theta_pend))./1.2e+1-(Lz_pend.^2.*m_pend.*cos(THE_Psi).*cos(THE_Theta).*cos(THE_Phi_pend).*cos(THE_Psi_pend).^2.*cos(THE_Theta_pend).*sin(THE_Theta_pend))./3.0-(Ly_pend.^2.*m_pend.*cos(THE_Theta).*cos(THE_Phi_pend).^2.*cos(THE_Psi_pend).*sin(THE_Psi).*sin(THE_Psi_pend).*sin(THE_Theta_pend))./6.0+Lz_pend.^2.*m_pend.*cos(THE_Theta).*cos(THE_Phi_pend).^2.*cos(THE_Psi_pend).*sin(THE_Psi).*sin(THE_Psi_pend).*sin(THE_Theta_pend).*(2.0./3.0)-(Ly_pend.^2.*m_pend.*cos(THE_Theta).*cos(THE_Phi_pend).*cos(THE_Psi_pend).^2.*cos(THE_Theta_pend).^2.*sin(THE_Psi).*sin(THE_Phi_pend))./1.2e+1+(Lz_pend.^2.*m_pend.*cos(THE_Theta).*cos(THE_Phi_pend).*cos(THE_Psi_pend).^2.*cos(THE_Theta_pend).^2.*sin(THE_Psi).*sin(THE_Phi_pend))./3.0+(Ly_pend.^2.*m_pend.*cos(THE_Psi).*cos(THE_Theta).*cos(THE_Psi_pend).*cos(THE_Theta_pend).*sin(THE_Phi_pend).*sin(THE_Psi_pend))./1.2e+1-(Lz_pend.^2.*m_pend.*cos(THE_Psi).*cos(THE_Theta).*cos(THE_Psi_pend).*cos(THE_Theta_pend).*sin(THE_Phi_pend).*sin(THE_Psi_pend))./3.0,I_xy.*cos(THE_Psi)+Iprop_xy.*cos(THE_Psi).*4.0-I_xz.*sin(THE_Psi)-Iprop_xz.*sin(THE_Psi).*4.0-(Ly_pend.^2.*m_pend.*cos(THE_Psi).*cos(THE_Phi_pend).*sin(THE_Phi_pend))./1.2e+1+(Lz_pend.^2.*m_pend.*cos(THE_Psi).*cos(THE_Phi_pend).*sin(THE_Phi_pend))./3.0-(Lx_pend.^2.*m_pend.*cos(THE_Phi_pend).*cos(THE_Theta_pend).*sin(THE_Psi).*sin(THE_Theta_pend))./1.2e+1+(Ly_pend.^2.*m_pend.*cos(THE_Psi).*cos(THE_Psi_pend).*sin(THE_Psi_pend).*sin(THE_Theta_pend))./1.2e+1+(Ly_pend.^2.*m_pend.*cos(THE_Phi_pend).*cos(THE_Theta_pend).*sin(THE_Psi).*sin(THE_Theta_pend))./1.2e+1-(Lz_pend.^2.*m_pend.*cos(THE_Psi).*cos(THE_Psi_pend).*sin(THE_Psi_pend).*sin(THE_Theta_pend))./3.0+(Lz_pend.*Tv_Z_pend.*m_pend.*sin(THE_Psi).*sin(THE_Phi_pend).*sin(THE_Psi_pend))./2.0-(Lx_pend.^2.*m_pend.*cos(THE_Psi).*cos(THE_Phi_pend).*cos(THE_Theta_pend).^2.*sin(THE_Phi_pend))./1.2e+1+(Ly_pend.^2.*m_pend.*cos(THE_Psi).*cos(THE_Phi_pend).*cos(THE_Psi_pend).^2.*sin(THE_Phi_pend))./6.0+(Ly_pend.^2.*m_pend.*cos(THE_Psi).*cos(THE_Phi_pend).*cos(THE_Theta_pend).^2.*sin(THE_Phi_pend))./1.2e+1-Lz_pend.^2.*m_pend.*cos(THE_Psi).*cos(THE_Phi_pend).*cos(THE_Psi_pend).^2.*sin(THE_Phi_pend).*(2.0./3.0)-(Ly_pend.^2.*m_pend.*cos(THE_Psi_pend).*cos(THE_Theta_pend).*sin(THE_Psi).*sin(THE_Phi_pend).*sin(THE_Psi_pend))./1.2e+1+(Lz_pend.^2.*m_pend.*cos(THE_Psi_pend).*cos(THE_Theta_pend).*sin(THE_Psi).*sin(THE_Phi_pend).*sin(THE_Psi_pend))./3.0+(Lz_pend.*Tv_Z_pend.*m_pend.*cos(THE_Phi_pend).*cos(THE_Psi_pend).*sin(THE_Psi).*sin(THE_Theta_pend))./2.0-(Ly_pend.^2.*m_pend.*cos(THE_Psi).*cos(THE_Phi_pend).^2.*cos(THE_Psi_pend).*sin(THE_Psi_pend).*sin(THE_Theta_pend))./6.0-(Ly_pend.^2.*m_pend.*cos(THE_Phi_pend).*cos(THE_Psi_pend).^2.*cos(THE_Theta_pend).*sin(THE_Psi).*sin(THE_Theta_pend))./1.2e+1+Lz_pend.^2.*m_pend.*cos(THE_Psi).*cos(THE_Phi_pend).^2.*cos(THE_Psi_pend).*sin(THE_Psi_pend).*sin(THE_Theta_pend).*(2.0./3.0)+(Lz_pend.^2.*m_pend.*cos(THE_Phi_pend).*cos(THE_Psi_pend).^2.*cos(THE_Theta_pend).*sin(THE_Psi).*sin(THE_Theta_pend))./3.0-(Ly_pend.^2.*m_pend.*cos(THE_Psi).*cos(THE_Phi_pend).*cos(THE_Psi_pend).^2.*cos(THE_Theta_pend).^2.*sin(THE_Phi_pend))./1.2e+1+(Lz_pend.^2.*m_pend.*cos(THE_Psi).*cos(THE_Phi_pend).*cos(THE_Psi_pend).^2.*cos(THE_Theta_pend).^2.*sin(THE_Phi_pend))./3.0,I_xx+Iprop_xx.*4.0+(Lx_pend.^2.*m_pend)./1.2e+1+(Ly_pend.^2.*m_pend)./1.2e+1+Tv_Z_pend.^2.*m_pend+cg_to_mot_H.^2.*mprop.*4.0+cg_to_mot_L.^2.*mprop.*2.0-(Ly_pend.^2.*m_pend.*cos(THE_Phi_pend).^2)./1.2e+1-(Ly_pend.^2.*m_pend.*cos(THE_Psi_pend).^2)./1.2e+1+(Lz_pend.^2.*m_pend.*cos(THE_Phi_pend).^2)./3.0+(Lz_pend.^2.*m_pend.*cos(THE_Psi_pend).^2)./3.0-(Lx_pend.^2.*m_pend.*cos(THE_Phi_pend).^2.*cos(THE_Theta_pend).^2)./1.2e+1+(Ly_pend.^2.*m_pend.*cos(THE_Phi_pend).^2.*cos(THE_Psi_pend).^2)./6.0+(Ly_pend.^2.*m_pend.*cos(THE_Phi_pend).^2.*cos(THE_Theta_pend).^2)./1.2e+1-Lz_pend.^2.*m_pend.*cos(THE_Phi_pend).^2.*cos(THE_Psi_pend).^2.*(2.0./3.0)-(Ly_pend.^2.*m_pend.*cos(THE_Phi_pend).^2.*cos(THE_Psi_pend).^2.*cos(THE_Theta_pend).^2)./1.2e+1+(Lz_pend.^2.*m_pend.*cos(THE_Phi_pend).^2.*cos(THE_Psi_pend).^2.*cos(THE_Theta_pend).^2)./3.0+Lz_pend.*Tv_Z_pend.*m_pend.*cos(THE_Psi_pend).*cos(THE_Theta_pend)+(Ly_pend.^2.*m_pend.*cos(THE_Phi_pend).*cos(THE_Psi_pend).*sin(THE_Phi_pend).*sin(THE_Psi_pend).*sin(THE_Theta_pend))./6.0-Lz_pend.^2.*m_pend.*cos(THE_Phi_pend).*cos(THE_Psi_pend).*sin(THE_Phi_pend).*sin(THE_Psi_pend).*sin(THE_Theta_pend).*(2.0./3.0),Tv_Z_pend.*m_pend.*cos(THE_Psi).*sin(THE_Phi)+cg_to_mot_H.*mprop.*cos(THE_Psi).*sin(THE_Phi).*4.0-Tv_Z_pend.*m_pend.*cos(THE_Phi).*sin(THE_Psi).*sin(THE_Theta)-cg_to_mot_H.*mprop.*cos(THE_Phi).*sin(THE_Psi).*sin(THE_Theta).*4.0+(Lz_pend.*m_pend.*cos(THE_Psi).*cos(THE_Psi_pend).*cos(THE_Theta_pend).*sin(THE_Phi))./2.0-(Lz_pend.*m_pend.*cos(THE_Phi_pend).*sin(THE_Phi).*sin(THE_Psi).*sin(THE_Psi_pend))./2.0-(Lz_pend.*m_pend.*cos(THE_Phi).*cos(THE_Psi).*cos(THE_Phi_pend).*sin(THE_Theta).*sin(THE_Psi_pend))./2.0-(Lz_pend.*m_pend.*cos(THE_Phi).*cos(THE_Psi_pend).*cos(THE_Theta_pend).*sin(THE_Psi).*sin(THE_Theta))./2.0+(Lz_pend.*m_pend.*cos(THE_Psi_pend).*sin(THE_Phi).*sin(THE_Psi).*sin(THE_Phi_pend).*sin(THE_Theta_pend))./2.0+(Lz_pend.*m_pend.*cos(THE_Phi).*cos(THE_Psi).*cos(THE_Psi_pend).*sin(THE_Theta).*sin(THE_Phi_pend).*sin(THE_Theta_pend))./2.0,-Tv_Z_pend.*m_pend.*cos(THE_Phi).*cos(THE_Psi)-cg_to_mot_H.*mprop.*cos(THE_Phi).*cos(THE_Psi).*4.0-Tv_Z_pend.*m_pend.*sin(THE_Phi).*sin(THE_Psi).*sin(THE_Theta)-cg_to_mot_H.*mprop.*sin(THE_Phi).*sin(THE_Psi).*sin(THE_Theta).*4.0+(Lz_pend.*m_pend.*cos(THE_Phi).*cos(THE_Phi_pend).*sin(THE_Psi).*sin(THE_Psi_pend))./2.0-(Lz_pend.*m_pend.*cos(THE_Phi).*cos(THE_Psi).*cos(THE_Psi_pend).*cos(THE_Theta_pend))./2.0-(Lz_pend.*m_pend.*cos(THE_Psi).*cos(THE_Phi_pend).*sin(THE_Phi).*sin(THE_Theta).*sin(THE_Psi_pend))./2.0-(Lz_pend.*m_pend.*cos(THE_Psi_pend).*cos(THE_Theta_pend).*sin(THE_Phi).*sin(THE_Psi).*sin(THE_Theta))./2.0-(Lz_pend.*m_pend.*cos(THE_Phi).*cos(THE_Psi_pend).*sin(THE_Psi).*sin(THE_Phi_pend).*sin(THE_Theta_pend))./2.0+(Lz_pend.*m_pend.*cos(THE_Psi).*cos(THE_Psi_pend).*sin(THE_Phi).*sin(THE_Theta).*sin(THE_Phi_pend).*sin(THE_Theta_pend))./2.0,cos(THE_Theta).*(Tv_Z_pend.*m_pend.*sin(THE_Psi).*2.0+cg_to_mot_H.*mprop.*sin(THE_Psi).*8.0+Lz_pend.*m_pend.*cos(THE_Psi).*cos(THE_Phi_pend).*sin(THE_Psi_pend)+Lz_pend.*m_pend.*cos(THE_Psi_pend).*cos(THE_Theta_pend).*sin(THE_Psi)-Lz_pend.*m_pend.*cos(THE_Psi).*cos(THE_Psi_pend).*sin(THE_Phi_pend).*sin(THE_Theta_pend)).*(-1.0./2.0),(Lx_pend.^2.*m_pend.*cos(THE_Phi_pend).*cos(THE_Theta_pend).*sin(THE_Theta_pend))./1.2e+1-(Ly_pend.^2.*m_pend.*cos(THE_Phi_pend).*cos(THE_Theta_pend).*sin(THE_Theta_pend))./1.2e+1-(Lz_pend.*Tv_Z_pend.*m_pend.*sin(THE_Phi_pend).*sin(THE_Psi_pend))./2.0+(Ly_pend.^2.*m_pend.*cos(THE_Psi_pend).*cos(THE_Theta_pend).*sin(THE_Phi_pend).*sin(THE_Psi_pend))./1.2e+1-(Lz_pend.^2.*m_pend.*cos(THE_Psi_pend).*cos(THE_Theta_pend).*sin(THE_Phi_pend).*sin(THE_Psi_pend))./3.0-(Lz_pend.*Tv_Z_pend.*m_pend.*cos(THE_Phi_pend).*cos(THE_Psi_pend).*sin(THE_Theta_pend))./2.0+(Ly_pend.^2.*m_pend.*cos(THE_Phi_pend).*cos(THE_Psi_pend).^2.*cos(THE_Theta_pend).*sin(THE_Theta_pend))./1.2e+1-(Lz_pend.^2.*m_pend.*cos(THE_Phi_pend).*cos(THE_Psi_pend).^2.*cos(THE_Theta_pend).*sin(THE_Theta_pend))./3.0,m_pend.*(Lx_pend.^2.*sin(THE_Phi_pend)+Ly_pend.^2.*sin(THE_Phi_pend)-Ly_pend.^2.*cos(THE_Psi_pend).^2.*sin(THE_Phi_pend)+Lz_pend.^2.*cos(THE_Psi_pend).^2.*sin(THE_Phi_pend).*4.0+Ly_pend.^2.*cos(THE_Phi_pend).*cos(THE_Psi_pend).*sin(THE_Psi_pend).*sin(THE_Theta_pend)-Lz_pend.^2.*cos(THE_Phi_pend).*cos(THE_Psi_pend).*sin(THE_Psi_pend).*sin(THE_Theta_pend).*4.0+Lz_pend.*Tv_Z_pend.*cos(THE_Psi_pend).*cos(THE_Theta_pend).*sin(THE_Phi_pend).*6.0).*(-1.0./1.2e+1),(m_pend.*(Ly_pend.^2.*cos(THE_Phi_pend).*cos(THE_Theta_pend)+Lz_pend.^2.*cos(THE_Phi_pend).*cos(THE_Theta_pend).*4.0+Lz_pend.*Tv_Z_pend.*cos(THE_Phi_pend).*cos(THE_Psi_pend).*6.0+Lz_pend.*Tv_Z_pend.*sin(THE_Phi_pend).*sin(THE_Psi_pend).*sin(THE_Theta_pend).*6.0))./1.2e+1,Tv_Z_pend.*m_pend.*cos(THE_Phi).*sin(THE_Psi)+cg_to_mot_H.*mprop.*cos(THE_Phi).*sin(THE_Psi).*4.0-Tv_Z_pend.*m_pend.*cos(THE_Psi).*sin(THE_Phi).*sin(THE_Theta)-cg_to_mot_H.*mprop.*cos(THE_Psi).*sin(THE_Phi).*sin(THE_Theta).*4.0+(Lz_pend.*m_pend.*cos(THE_Phi).*cos(THE_Psi).*cos(THE_Phi_pend).*sin(THE_Psi_pend))./2.0+(Lz_pend.*m_pend.*cos(THE_Phi).*cos(THE_Psi_pend).*cos(THE_Theta_pend).*sin(THE_Psi))./2.0-(Lz_pend.*m_pend.*cos(THE_Theta).*sin(THE_Phi).*sin(THE_Phi_pend).*sin(THE_Psi_pend))./2.0-(Lz_pend.*m_pend.*cos(THE_Psi).*cos(THE_Psi_pend).*cos(THE_Theta_pend).*sin(THE_Phi).*sin(THE_Theta))./2.0-(Lz_pend.*m_pend.*cos(THE_Phi).*cos(THE_Psi).*cos(THE_Psi_pend).*sin(THE_Phi_pend).*sin(THE_Theta_pend))./2.0-(Lz_pend.*m_pend.*cos(THE_Theta).*cos(THE_Phi_pend).*cos(THE_Psi_pend).*sin(THE_Phi).*sin(THE_Theta_pend))./2.0+(Lz_pend.*m_pend.*cos(THE_Phi_pend).*sin(THE_Phi).*sin(THE_Psi).*sin(THE_Theta).*sin(THE_Psi_pend))./2.0-(Lz_pend.*m_pend.*cos(THE_Psi_pend).*sin(THE_Phi).*sin(THE_Psi).*sin(THE_Theta).*sin(THE_Phi_pend).*sin(THE_Theta_pend))./2.0,(cos(THE_Phi).*(Tv_Z_pend.*m_pend.*cos(THE_Psi).*cos(THE_Theta).*2.0+cg_to_mot_H.*mprop.*cos(THE_Psi).*cos(THE_Theta).*8.0-Lz_pend.*m_pend.*sin(THE_Theta).*sin(THE_Phi_pend).*sin(THE_Psi_pend)-Lz_pend.*m_pend.*cos(THE_Theta).*cos(THE_Phi_pend).*sin(THE_Psi).*sin(THE_Psi_pend)-Lz_pend.*m_pend.*cos(THE_Phi_pend).*cos(THE_Psi_pend).*sin(THE_Theta).*sin(THE_Theta_pend)+Lz_pend.*m_pend.*cos(THE_Psi).*cos(THE_Theta).*cos(THE_Psi_pend).*cos(THE_Theta_pend)+Lz_pend.*m_pend.*cos(THE_Theta).*cos(THE_Psi_pend).*sin(THE_Psi).*sin(THE_Phi_pend).*sin(THE_Theta_pend)))./2.0,Tv_Z_pend.*m_pend.*cos(THE_Psi).*sin(THE_Phi)+cg_to_mot_H.*mprop.*cos(THE_Psi).*sin(THE_Phi).*4.0-Tv_Z_pend.*m_pend.*cos(THE_Phi).*sin(THE_Psi).*sin(THE_Theta)-cg_to_mot_H.*mprop.*cos(THE_Phi).*sin(THE_Psi).*sin(THE_Theta).*4.0+(Lz_pend.*m_pend.*cos(THE_Psi).*cos(THE_Psi_pend).*cos(THE_Theta_pend).*sin(THE_Phi))./2.0-(Lz_pend.*m_pend.*cos(THE_Phi_pend).*sin(THE_Phi).*sin(THE_Psi).*sin(THE_Psi_pend))./2.0-(Lz_pend.*m_pend.*cos(THE_Phi).*cos(THE_Psi).*cos(THE_Phi_pend).*sin(THE_Theta).*sin(THE_Psi_pend))./2.0-(Lz_pend.*m_pend.*cos(THE_Phi).*cos(THE_Psi_pend).*cos(THE_Theta_pend).*sin(THE_Psi).*sin(THE_Theta))./2.0+(Lz_pend.*m_pend.*cos(THE_Psi_pend).*sin(THE_Phi).*sin(THE_Psi).*sin(THE_Phi_pend).*sin(THE_Theta_pend))./2.0+(Lz_pend.*m_pend.*cos(THE_Phi).*cos(THE_Psi).*cos(THE_Psi_pend).*sin(THE_Theta).*sin(THE_Phi_pend).*sin(THE_Theta_pend))./2.0,m+m_pend+mprop.*4.0,0.0,0.0,(Lz_pend.*m_pend.*(cos(THE_Phi).*cos(THE_Theta).*cos(THE_Phi_pend).*sin(THE_Psi_pend)-cos(THE_Psi).*sin(THE_Phi).*sin(THE_Phi_pend).*sin(THE_Psi_pend)-cos(THE_Psi).*cos(THE_Phi_pend).*cos(THE_Psi_pend).*sin(THE_Phi).*sin(THE_Theta_pend)-cos(THE_Phi).*cos(THE_Theta).*cos(THE_Psi_pend).*sin(THE_Phi_pend).*sin(THE_Theta_pend)+cos(THE_Phi).*sin(THE_Psi).*sin(THE_Theta).*sin(THE_Phi_pend).*sin(THE_Psi_pend)+cos(THE_Phi).*cos(THE_Phi_pend).*cos(THE_Psi_pend).*sin(THE_Psi).*sin(THE_Theta).*sin(THE_Theta_pend)))./2.0,Lz_pend.*m_pend.*cos(THE_Psi_pend).*(sin(THE_Phi).*sin(THE_Psi).*sin(THE_Theta_pend)-cos(THE_Phi).*cos(THE_Theta).*cos(THE_Phi_pend).*cos(THE_Theta_pend)+cos(THE_Phi).*cos(THE_Psi).*sin(THE_Theta).*sin(THE_Theta_pend)+cos(THE_Psi).*cos(THE_Theta_pend).*sin(THE_Phi).*sin(THE_Phi_pend)-cos(THE_Phi).*cos(THE_Theta_pend).*sin(THE_Psi).*sin(THE_Theta).*sin(THE_Phi_pend)).*(-1.0./2.0),Lz_pend.*m_pend.*(-cos(THE_Psi).*cos(THE_Phi_pend).*cos(THE_Psi_pend).*sin(THE_Phi)-cos(THE_Phi).*cos(THE_Theta).*cos(THE_Psi_pend).*sin(THE_Phi_pend)+cos(THE_Theta_pend).*sin(THE_Phi).*sin(THE_Psi).*sin(THE_Psi_pend)+cos(THE_Phi).*cos(THE_Phi_pend).*cos(THE_Psi_pend).*sin(THE_Psi).*sin(THE_Theta)+cos(THE_Phi).*cos(THE_Psi).*cos(THE_Theta_pend).*sin(THE_Theta).*sin(THE_Psi_pend)+cos(THE_Phi).*cos(THE_Theta).*cos(THE_Phi_pend).*sin(THE_Psi_pend).*sin(THE_Theta_pend)-cos(THE_Psi).*sin(THE_Phi).*sin(THE_Phi_pend).*sin(THE_Psi_pend).*sin(THE_Theta_pend)+cos(THE_Phi).*sin(THE_Psi).*sin(THE_Theta).*sin(THE_Phi_pend).*sin(THE_Psi_pend).*sin(THE_Theta_pend)).*(-1.0./2.0),Tv_Z_pend.*m_pend.*sin(THE_Phi).*sin(THE_Psi)+cg_to_mot_H.*mprop.*sin(THE_Phi).*sin(THE_Psi).*4.0+Tv_Z_pend.*m_pend.*cos(THE_Phi).*cos(THE_Psi).*sin(THE_Theta)+cg_to_mot_H.*mprop.*cos(THE_Phi).*cos(THE_Psi).*sin(THE_Theta).*4.0+(Lz_pend.*m_pend.*cos(THE_Psi).*cos(THE_Phi_pend).*sin(THE_Phi).*sin(THE_Psi_pend))./2.0+(Lz_pend.*m_pend.*cos(THE_Phi).*cos(THE_Theta).*sin(THE_Phi_pend).*sin(THE_Psi_pend))./2.0+(Lz_pend.*m_pend.*cos(THE_Psi_pend).*cos(THE_Theta_pend).*sin(THE_Phi).*sin(THE_Psi))./2.0+(Lz_pend.*m_pend.*cos(THE_Phi).*cos(THE_Psi).*cos(THE_Psi_pend).*cos(THE_Theta_pend).*sin(THE_Theta))./2.0+(Lz_pend.*m_pend.*cos(THE_Phi).*cos(THE_Theta).*cos(THE_Phi_pend).*cos(THE_Psi_pend).*sin(THE_Theta_pend))./2.0-(Lz_pend.*m_pend.*cos(THE_Phi).*cos(THE_Phi_pend).*sin(THE_Psi).*sin(THE_Theta).*sin(THE_Psi_pend))./2.0-(Lz_pend.*m_pend.*cos(THE_Psi).*cos(THE_Psi_pend).*sin(THE_Phi).*sin(THE_Phi_pend).*sin(THE_Theta_pend))./2.0+(Lz_pend.*m_pend.*cos(THE_Phi).*cos(THE_Psi_pend).*sin(THE_Psi).*sin(THE_Theta).*sin(THE_Phi_pend).*sin(THE_Theta_pend))./2.0,(sin(THE_Phi).*(Tv_Z_pend.*m_pend.*cos(THE_Psi).*cos(THE_Theta).*2.0+cg_to_mot_H.*mprop.*cos(THE_Psi).*cos(THE_Theta).*8.0-Lz_pend.*m_pend.*sin(THE_Theta).*sin(THE_Phi_pend).*sin(THE_Psi_pend)-Lz_pend.*m_pend.*cos(THE_Theta).*cos(THE_Phi_pend).*sin(THE_Psi).*sin(THE_Psi_pend)-Lz_pend.*m_pend.*cos(THE_Phi_pend).*cos(THE_Psi_pend).*sin(THE_Theta).*sin(THE_Theta_pend)+Lz_pend.*m_pend.*cos(THE_Psi).*cos(THE_Theta).*cos(THE_Psi_pend).*cos(THE_Theta_pend)+Lz_pend.*m_pend.*cos(THE_Theta).*cos(THE_Psi_pend).*sin(THE_Psi).*sin(THE_Phi_pend).*sin(THE_Theta_pend)))./2.0,-Tv_Z_pend.*m_pend.*cos(THE_Phi).*cos(THE_Psi)-cg_to_mot_H.*mprop.*cos(THE_Phi).*cos(THE_Psi).*4.0-Tv_Z_pend.*m_pend.*sin(THE_Phi).*sin(THE_Psi).*sin(THE_Theta)-cg_to_mot_H.*mprop.*sin(THE_Phi).*sin(THE_Psi).*sin(THE_Theta).*4.0+(Lz_pend.*m_pend.*cos(THE_Phi).*cos(THE_Phi_pend).*sin(THE_Psi).*sin(THE_Psi_pend))./2.0-(Lz_pend.*m_pend.*cos(THE_Phi).*cos(THE_Psi).*cos(THE_Psi_pend).*cos(THE_Theta_pend))./2.0-(Lz_pend.*m_pend.*cos(THE_Psi).*cos(THE_Phi_pend).*sin(THE_Phi).*sin(THE_Theta).*sin(THE_Psi_pend))./2.0-(Lz_pend.*m_pend.*cos(THE_Psi_pend).*cos(THE_Theta_pend).*sin(THE_Phi).*sin(THE_Psi).*sin(THE_Theta))./2.0-(Lz_pend.*m_pend.*cos(THE_Phi).*cos(THE_Psi_pend).*sin(THE_Psi).*sin(THE_Phi_pend).*sin(THE_Theta_pend))./2.0+(Lz_pend.*m_pend.*cos(THE_Psi).*cos(THE_Psi_pend).*sin(THE_Phi).*sin(THE_Theta).*sin(THE_Phi_pend).*sin(THE_Theta_pend))./2.0,0.0,m+m_pend+mprop.*4.0,0.0,(Lz_pend.*m_pend.*(cos(THE_Phi).*cos(THE_Psi).*sin(THE_Phi_pend).*sin(THE_Psi_pend)+cos(THE_Theta).*cos(THE_Phi_pend).*sin(THE_Phi).*sin(THE_Psi_pend)+cos(THE_Phi).*cos(THE_Psi).*cos(THE_Phi_pend).*cos(THE_Psi_pend).*sin(THE_Theta_pend)-cos(THE_Theta).*cos(THE_Psi_pend).*sin(THE_Phi).*sin(THE_Phi_pend).*sin(THE_Theta_pend)+sin(THE_Phi).*sin(THE_Psi).*sin(THE_Theta).*sin(THE_Phi_pend).*sin(THE_Psi_pend)+cos(THE_Phi_pend).*cos(THE_Psi_pend).*sin(THE_Phi).*sin(THE_Psi).*sin(THE_Theta).*sin(THE_Theta_pend)))./2.0,(Lz_pend.*m_pend.*cos(THE_Psi_pend).*(cos(THE_Phi).*sin(THE_Psi).*sin(THE_Theta_pend)+cos(THE_Phi).*cos(THE_Psi).*cos(THE_Theta_pend).*sin(THE_Phi_pend)+cos(THE_Theta).*cos(THE_Phi_pend).*cos(THE_Theta_pend).*sin(THE_Phi)-cos(THE_Psi).*sin(THE_Phi).*sin(THE_Theta).*sin(THE_Theta_pend)+cos(THE_Theta_pend).*sin(THE_Phi).*sin(THE_Psi).*sin(THE_Theta).*sin(THE_Phi_pend)))./2.0,Lz_pend.*m_pend.*(cos(THE_Phi).*cos(THE_Psi).*cos(THE_Phi_pend).*cos(THE_Psi_pend)-cos(THE_Theta).*cos(THE_Psi_pend).*sin(THE_Phi).*sin(THE_Phi_pend)-cos(THE_Phi).*cos(THE_Theta_pend).*sin(THE_Psi).*sin(THE_Psi_pend)+cos(THE_Phi_pend).*cos(THE_Psi_pend).*sin(THE_Phi).*sin(THE_Psi).*sin(THE_Theta)+cos(THE_Psi).*cos(THE_Theta_pend).*sin(THE_Phi).*sin(THE_Theta).*sin(THE_Psi_pend)+cos(THE_Phi).*cos(THE_Psi).*sin(THE_Phi_pend).*sin(THE_Psi_pend).*sin(THE_Theta_pend)+cos(THE_Theta).*cos(THE_Phi_pend).*sin(THE_Phi).*sin(THE_Psi_pend).*sin(THE_Theta_pend)+sin(THE_Phi).*sin(THE_Psi).*sin(THE_Theta).*sin(THE_Phi_pend).*sin(THE_Psi_pend).*sin(THE_Theta_pend)).*(-1.0./2.0),0.0,-Tv_Z_pend.*m_pend.*cos(THE_Psi).*sin(THE_Theta)-cg_to_mot_H.*mprop.*cos(THE_Psi).*sin(THE_Theta).*4.0-(Lz_pend.*m_pend.*cos(THE_Theta).*sin(THE_Phi_pend).*sin(THE_Psi_pend))./2.0-(Lz_pend.*m_pend.*cos(THE_Psi).*cos(THE_Psi_pend).*cos(THE_Theta_pend).*sin(THE_Theta))./2.0-(Lz_pend.*m_pend.*cos(THE_Theta).*cos(THE_Phi_pend).*cos(THE_Psi_pend).*sin(THE_Theta_pend))./2.0+(Lz_pend.*m_pend.*cos(THE_Phi_pend).*sin(THE_Psi).*sin(THE_Theta).*sin(THE_Psi_pend))./2.0-(Lz_pend.*m_pend.*cos(THE_Psi_pend).*sin(THE_Psi).*sin(THE_Theta).*sin(THE_Phi_pend).*sin(THE_Theta_pend))./2.0,cos(THE_Theta).*(Tv_Z_pend.*m_pend.*sin(THE_Psi).*2.0+cg_to_mot_H.*mprop.*sin(THE_Psi).*8.0+Lz_pend.*m_pend.*cos(THE_Psi).*cos(THE_Phi_pend).*sin(THE_Psi_pend)+Lz_pend.*m_pend.*cos(THE_Psi_pend).*cos(THE_Theta_pend).*sin(THE_Psi)-Lz_pend.*m_pend.*cos(THE_Psi).*cos(THE_Psi_pend).*sin(THE_Phi_pend).*sin(THE_Theta_pend)).*(-1.0./2.0),0.0,0.0,m+m_pend+mprop.*4.0,(Lz_pend.*m_pend.*(-cos(THE_Phi_pend).*sin(THE_Theta).*sin(THE_Psi_pend)+cos(THE_Theta).*sin(THE_Psi).*sin(THE_Phi_pend).*sin(THE_Psi_pend)+cos(THE_Psi_pend).*sin(THE_Theta).*sin(THE_Phi_pend).*sin(THE_Theta_pend)+cos(THE_Theta).*cos(THE_Phi_pend).*cos(THE_Psi_pend).*sin(THE_Psi).*sin(THE_Theta_pend)))./2.0,Lz_pend.*m_pend.*cos(THE_Psi_pend).*(cos(THE_Psi).*cos(THE_Theta).*sin(THE_Theta_pend)+cos(THE_Phi_pend).*cos(THE_Theta_pend).*sin(THE_Theta)-cos(THE_Theta).*cos(THE_Theta_pend).*sin(THE_Psi).*sin(THE_Phi_pend)).*(-1.0./2.0),Lz_pend.*m_pend.*(cos(THE_Psi_pend).*sin(THE_Theta).*sin(THE_Phi_pend)+cos(THE_Theta).*cos(THE_Phi_pend).*cos(THE_Psi_pend).*sin(THE_Psi)+cos(THE_Psi).*cos(THE_Theta).*cos(THE_Theta_pend).*sin(THE_Psi_pend)-cos(THE_Phi_pend).*sin(THE_Theta).*sin(THE_Psi_pend).*sin(THE_Theta_pend)+cos(THE_Theta).*sin(THE_Psi).*sin(THE_Phi_pend).*sin(THE_Psi_pend).*sin(THE_Theta_pend)).*(-1.0./2.0),(Ly_pend.^2.*m_pend.*cos(THE_Psi).*cos(THE_Theta))./1.2e+1+(Lz_pend.^2.*m_pend.*cos(THE_Psi).*cos(THE_Theta))./3.0+(Lx_pend.^2.*m_pend.*cos(THE_Psi).*cos(THE_Theta).*cos(THE_Theta_pend).^2)./1.2e+1-(Ly_pend.^2.*m_pend.*cos(THE_Psi).*cos(THE_Theta).*cos(THE_Theta_pend).^2)./1.2e+1+(Ly_pend.^2.*m_pend.*cos(THE_Psi).*cos(THE_Theta).*cos(THE_Psi_pend).^2.*cos(THE_Theta_pend).^2)./1.2e+1-(Lz_pend.^2.*m_pend.*cos(THE_Psi).*cos(THE_Theta).*cos(THE_Psi_pend).^2.*cos(THE_Theta_pend).^2)./3.0-(Lx_pend.^2.*m_pend.*cos(THE_Phi_pend).*cos(THE_Theta_pend).*sin(THE_Theta).*sin(THE_Theta_pend))./1.2e+1+(Ly_pend.^2.*m_pend.*cos(THE_Phi_pend).*cos(THE_Theta_pend).*sin(THE_Theta).*sin(THE_Theta_pend))./1.2e+1+(Lz_pend.*Tv_Z_pend.*m_pend.*sin(THE_Theta).*sin(THE_Phi_pend).*sin(THE_Psi_pend))./2.0+(Lx_pend.^2.*m_pend.*cos(THE_Theta).*cos(THE_Theta_pend).*sin(THE_Psi).*sin(THE_Phi_pend).*sin(THE_Theta_pend))./1.2e+1-(Ly_pend.^2.*m_pend.*cos(THE_Theta).*cos(THE_Theta_pend).*sin(THE_Psi).*sin(THE_Phi_pend).*sin(THE_Theta_pend))./1.2e+1-(Ly_pend.^2.*m_pend.*cos(THE_Psi_pend).*cos(THE_Theta_pend).*sin(THE_Theta).*sin(THE_Phi_pend).*sin(THE_Psi_pend))./1.2e+1+(Lz_pend.^2.*m_pend.*cos(THE_Psi_pend).*cos(THE_Theta_pend).*sin(THE_Theta).*sin(THE_Phi_pend).*sin(THE_Psi_pend))./3.0+(Lz_pend.*Tv_Z_pend.*m_pend.*cos(THE_Theta).*cos(THE_Phi_pend).*sin(THE_Psi).*sin(THE_Psi_pend))./2.0+(Lz_pend.*Tv_Z_pend.*m_pend.*cos(THE_Phi_pend).*cos(THE_Psi_pend).*sin(THE_Theta).*sin(THE_Theta_pend))./2.0-(Ly_pend.^2.*m_pend.*cos(THE_Phi_pend).*cos(THE_Psi_pend).^2.*cos(THE_Theta_pend).*sin(THE_Theta).*sin(THE_Theta_pend))./1.2e+1+(Lz_pend.^2.*m_pend.*cos(THE_Phi_pend).*cos(THE_Psi_pend).^2.*cos(THE_Theta_pend).*sin(THE_Theta).*sin(THE_Theta_pend))./3.0-(Lz_pend.*Tv_Z_pend.*m_pend.*cos(THE_Theta).*cos(THE_Psi_pend).*sin(THE_Psi).*sin(THE_Phi_pend).*sin(THE_Theta_pend))./2.0+(Ly_pend.^2.*m_pend.*cos(THE_Theta).*cos(THE_Psi_pend).^2.*cos(THE_Theta_pend).*sin(THE_Psi).*sin(THE_Phi_pend).*sin(THE_Theta_pend))./1.2e+1-(Lz_pend.^2.*m_pend.*cos(THE_Theta).*cos(THE_Psi_pend).^2.*cos(THE_Theta_pend).*sin(THE_Psi).*sin(THE_Phi_pend).*sin(THE_Theta_pend))./3.0-(Ly_pend.^2.*m_pend.*cos(THE_Theta).*cos(THE_Phi_pend).*cos(THE_Psi_pend).*cos(THE_Theta_pend).*sin(THE_Psi).*sin(THE_Psi_pend))./1.2e+1+(Lz_pend.^2.*m_pend.*cos(THE_Theta).*cos(THE_Phi_pend).*cos(THE_Psi_pend).*cos(THE_Theta_pend).*sin(THE_Psi).*sin(THE_Psi_pend))./3.0,Ly_pend.^2.*m_pend.*sin(THE_Psi).*(-1.0./1.2e+1)-(Lz_pend.^2.*m_pend.*sin(THE_Psi))./3.0-(Lx_pend.^2.*m_pend.*cos(THE_Theta_pend).^2.*sin(THE_Psi))./1.2e+1+(Ly_pend.^2.*m_pend.*cos(THE_Theta_pend).^2.*sin(THE_Psi))./1.2e+1-(Ly_pend.^2.*m_pend.*cos(THE_Psi_pend).^2.*cos(THE_Theta_pend).^2.*sin(THE_Psi))./1.2e+1+(Lz_pend.^2.*m_pend.*cos(THE_Psi_pend).^2.*cos(THE_Theta_pend).^2.*sin(THE_Psi))./3.0+(Lx_pend.^2.*m_pend.*cos(THE_Psi).*cos(THE_Theta_pend).*sin(THE_Phi_pend).*sin(THE_Theta_pend))./1.2e+1-(Ly_pend.^2.*m_pend.*cos(THE_Psi).*cos(THE_Theta_pend).*sin(THE_Phi_pend).*sin(THE_Theta_pend))./1.2e+1+(Lz_pend.*Tv_Z_pend.*m_pend.*cos(THE_Psi).*cos(THE_Phi_pend).*sin(THE_Psi_pend))./2.0-(Ly_pend.^2.*m_pend.*cos(THE_Psi).*cos(THE_Phi_pend).*cos(THE_Psi_pend).*cos(THE_Theta_pend).*sin(THE_Psi_pend))./1.2e+1+(Lz_pend.^2.*m_pend.*cos(THE_Psi).*cos(THE_Phi_pend).*cos(THE_Psi_pend).*cos(THE_Theta_pend).*sin(THE_Psi_pend))./3.0-(Lz_pend.*Tv_Z_pend.*m_pend.*cos(THE_Psi).*cos(THE_Psi_pend).*sin(THE_Phi_pend).*sin(THE_Theta_pend))./2.0+(Ly_pend.^2.*m_pend.*cos(THE_Psi).*cos(THE_Psi_pend).^2.*cos(THE_Theta_pend).*sin(THE_Phi_pend).*sin(THE_Theta_pend))./1.2e+1-(Lz_pend.^2.*m_pend.*cos(THE_Psi).*cos(THE_Psi_pend).^2.*cos(THE_Theta_pend).*sin(THE_Phi_pend).*sin(THE_Theta_pend))./3.0,(Lx_pend.^2.*m_pend.*cos(THE_Phi_pend).*cos(THE_Theta_pend).*sin(THE_Theta_pend))./1.2e+1-(Ly_pend.^2.*m_pend.*cos(THE_Phi_pend).*cos(THE_Theta_pend).*sin(THE_Theta_pend))./1.2e+1-(Lz_pend.*Tv_Z_pend.*m_pend.*sin(THE_Phi_pend).*sin(THE_Psi_pend))./2.0+(Ly_pend.^2.*m_pend.*cos(THE_Psi_pend).*cos(THE_Theta_pend).*sin(THE_Phi_pend).*sin(THE_Psi_pend))./1.2e+1-(Lz_pend.^2.*m_pend.*cos(THE_Psi_pend).*cos(THE_Theta_pend).*sin(THE_Phi_pend).*sin(THE_Psi_pend))./3.0-(Lz_pend.*Tv_Z_pend.*m_pend.*cos(THE_Phi_pend).*cos(THE_Psi_pend).*sin(THE_Theta_pend))./2.0+(Ly_pend.^2.*m_pend.*cos(THE_Phi_pend).*cos(THE_Psi_pend).^2.*cos(THE_Theta_pend).*sin(THE_Theta_pend))./1.2e+1-(Lz_pend.^2.*m_pend.*cos(THE_Phi_pend).*cos(THE_Psi_pend).^2.*cos(THE_Theta_pend).*sin(THE_Theta_pend))./3.0,(Lz_pend.*m_pend.*(cos(THE_Phi).*cos(THE_Theta).*cos(THE_Phi_pend).*sin(THE_Psi_pend)-cos(THE_Psi).*sin(THE_Phi).*sin(THE_Phi_pend).*sin(THE_Psi_pend)-cos(THE_Psi).*cos(THE_Phi_pend).*cos(THE_Psi_pend).*sin(THE_Phi).*sin(THE_Theta_pend)-cos(THE_Phi).*cos(THE_Theta).*cos(THE_Psi_pend).*sin(THE_Phi_pend).*sin(THE_Theta_pend)+cos(THE_Phi).*sin(THE_Psi).*sin(THE_Theta).*sin(THE_Phi_pend).*sin(THE_Psi_pend)+cos(THE_Phi).*cos(THE_Phi_pend).*cos(THE_Psi_pend).*sin(THE_Psi).*sin(THE_Theta).*sin(THE_Theta_pend)))./2.0,(Lz_pend.*m_pend.*(cos(THE_Phi).*cos(THE_Psi).*sin(THE_Phi_pend).*sin(THE_Psi_pend)+cos(THE_Theta).*cos(THE_Phi_pend).*sin(THE_Phi).*sin(THE_Psi_pend)+cos(THE_Phi).*cos(THE_Psi).*cos(THE_Phi_pend).*cos(THE_Psi_pend).*sin(THE_Theta_pend)-cos(THE_Theta).*cos(THE_Psi_pend).*sin(THE_Phi).*sin(THE_Phi_pend).*sin(THE_Theta_pend)+sin(THE_Phi).*sin(THE_Psi).*sin(THE_Theta).*sin(THE_Phi_pend).*sin(THE_Psi_pend)+cos(THE_Phi_pend).*cos(THE_Psi_pend).*sin(THE_Phi).*sin(THE_Psi).*sin(THE_Theta).*sin(THE_Theta_pend)))./2.0,(Lz_pend.*m_pend.*(-cos(THE_Phi_pend).*sin(THE_Theta).*sin(THE_Psi_pend)+cos(THE_Theta).*sin(THE_Psi).*sin(THE_Phi_pend).*sin(THE_Psi_pend)+cos(THE_Psi_pend).*sin(THE_Theta).*sin(THE_Phi_pend).*sin(THE_Theta_pend)+cos(THE_Theta).*cos(THE_Phi_pend).*cos(THE_Psi_pend).*sin(THE_Psi).*sin(THE_Theta_pend)))./2.0,(m_pend.*(-Lx_pend.^2.*sin(THE_Theta_pend).^2-Ly_pend.^2.*sin(THE_Psi_pend).^2+Lz_pend.^2.*sin(THE_Psi_pend).^2.*4.0+Lz_pend.^2.*sin(THE_Theta_pend).^2.*4.0+Lx_pend.^2+Ly_pend.^2+Ly_pend.^2.*sin(THE_Psi_pend).^2.*sin(THE_Theta_pend).^2-Lz_pend.^2.*sin(THE_Psi_pend).^2.*sin(THE_Theta_pend).^2.*4.0))./1.2e+1,m_pend.*cos(THE_Psi_pend).*cos(THE_Theta_pend).*sin(THE_Psi_pend).*(Ly_pend.^2-Lz_pend.^2.*4.0).*(-1.0./1.2e+1),m_pend.*sin(THE_Theta_pend).*(Ly_pend.^2+Lz_pend.^2.*4.0).*(-1.0./1.2e+1),(Lx_pend.^2.*m_pend.*sin(THE_Theta).*sin(THE_Phi_pend))./1.2e+1+(Ly_pend.^2.*m_pend.*sin(THE_Theta).*sin(THE_Phi_pend))./1.2e+1-(Ly_pend.^2.*m_pend.*cos(THE_Psi_pend).^2.*sin(THE_Theta).*sin(THE_Phi_pend))./1.2e+1+(Lz_pend.^2.*m_pend.*cos(THE_Psi_pend).^2.*sin(THE_Theta).*sin(THE_Phi_pend))./3.0+(Lx_pend.^2.*m_pend.*cos(THE_Theta).*cos(THE_Phi_pend).*sin(THE_Psi))./1.2e+1+(Ly_pend.^2.*m_pend.*cos(THE_Theta).*cos(THE_Phi_pend).*sin(THE_Psi))./1.2e+1-(Ly_pend.^2.*m_pend.*cos(THE_Theta).*cos(THE_Phi_pend).*cos(THE_Psi_pend).^2.*sin(THE_Psi))./1.2e+1+(Lz_pend.^2.*m_pend.*cos(THE_Theta).*cos(THE_Phi_pend).*cos(THE_Psi_pend).^2.*sin(THE_Psi))./3.0-(Ly_pend.^2.*m_pend.*cos(THE_Psi).*cos(THE_Theta).*cos(THE_Psi_pend).*cos(THE_Theta_pend).*sin(THE_Psi_pend))./1.2e+1+(Lz_pend.^2.*m_pend.*cos(THE_Psi).*cos(THE_Theta).*cos(THE_Psi_pend).*cos(THE_Theta_pend).*sin(THE_Psi_pend))./3.0+(Ly_pend.^2.*m_pend.*cos(THE_Phi_pend).*cos(THE_Psi_pend).*sin(THE_Theta).*sin(THE_Psi_pend).*sin(THE_Theta_pend))./1.2e+1-(Lz_pend.^2.*m_pend.*cos(THE_Phi_pend).*cos(THE_Psi_pend).*sin(THE_Theta).*sin(THE_Psi_pend).*sin(THE_Theta_pend))./3.0+(Lz_pend.*Tv_Z_pend.*m_pend.*cos(THE_Psi_pend).*cos(THE_Theta_pend).*sin(THE_Theta).*sin(THE_Phi_pend))./2.0-(Ly_pend.^2.*m_pend.*cos(THE_Theta).*cos(THE_Psi_pend).*sin(THE_Psi).*sin(THE_Phi_pend).*sin(THE_Psi_pend).*sin(THE_Theta_pend))./1.2e+1+(Lz_pend.^2.*m_pend.*cos(THE_Theta).*cos(THE_Psi_pend).*sin(THE_Psi).*sin(THE_Phi_pend).*sin(THE_Psi_pend).*sin(THE_Theta_pend))./3.0+(Lz_pend.*Tv_Z_pend.*m_pend.*cos(THE_Theta).*cos(THE_Phi_pend).*cos(THE_Psi_pend).*cos(THE_Theta_pend).*sin(THE_Psi))./2.0,(Lx_pend.^2.*m_pend.*cos(THE_Psi).*cos(THE_Phi_pend))./1.2e+1+(Ly_pend.^2.*m_pend.*cos(THE_Psi).*cos(THE_Phi_pend))./1.2e+1-(Ly_pend.^2.*m_pend.*cos(THE_Psi).*cos(THE_Phi_pend).*cos(THE_Psi_pend).^2)./1.2e+1+(Lz_pend.^2.*m_pend.*cos(THE_Psi).*cos(THE_Phi_pend).*cos(THE_Psi_pend).^2)./3.0+(Ly_pend.^2.*m_pend.*cos(THE_Psi_pend).*cos(THE_Theta_pend).*sin(THE_Psi).*sin(THE_Psi_pend))./1.2e+1-(Lz_pend.^2.*m_pend.*cos(THE_Psi_pend).*cos(THE_Theta_pend).*sin(THE_Psi).*sin(THE_Psi_pend))./3.0-(Ly_pend.^2.*m_pend.*cos(THE_Psi).*cos(THE_Psi_pend).*sin(THE_Phi_pend).*sin(THE_Psi_pend).*sin(THE_Theta_pend))./1.2e+1+(Lz_pend.^2.*m_pend.*cos(THE_Psi).*cos(THE_Psi_pend).*sin(THE_Phi_pend).*sin(THE_Psi_pend).*sin(THE_Theta_pend))./3.0+(Lz_pend.*Tv_Z_pend.*m_pend.*cos(THE_Psi).*cos(THE_Phi_pend).*cos(THE_Psi_pend).*cos(THE_Theta_pend))./2.0,m_pend.*(Lx_pend.^2.*sin(THE_Phi_pend)+Ly_pend.^2.*sin(THE_Phi_pend)-Ly_pend.^2.*cos(THE_Psi_pend).^2.*sin(THE_Phi_pend)+Lz_pend.^2.*cos(THE_Psi_pend).^2.*sin(THE_Phi_pend).*4.0+Ly_pend.^2.*cos(THE_Phi_pend).*cos(THE_Psi_pend).*sin(THE_Psi_pend).*sin(THE_Theta_pend)-Lz_pend.^2.*cos(THE_Phi_pend).*cos(THE_Psi_pend).*sin(THE_Psi_pend).*sin(THE_Theta_pend).*4.0+Lz_pend.*Tv_Z_pend.*cos(THE_Psi_pend).*cos(THE_Theta_pend).*sin(THE_Phi_pend).*6.0).*(-1.0./1.2e+1),Lz_pend.*m_pend.*cos(THE_Psi_pend).*(sin(THE_Phi).*sin(THE_Psi).*sin(THE_Theta_pend)-cos(THE_Phi).*cos(THE_Theta).*cos(THE_Phi_pend).*cos(THE_Theta_pend)+cos(THE_Phi).*cos(THE_Psi).*sin(THE_Theta).*sin(THE_Theta_pend)+cos(THE_Psi).*cos(THE_Theta_pend).*sin(THE_Phi).*sin(THE_Phi_pend)-cos(THE_Phi).*cos(THE_Theta_pend).*sin(THE_Psi).*sin(THE_Theta).*sin(THE_Phi_pend)).*(-1.0./2.0),(Lz_pend.*m_pend.*cos(THE_Psi_pend).*(cos(THE_Phi).*sin(THE_Psi).*sin(THE_Theta_pend)+cos(THE_Phi).*cos(THE_Psi).*cos(THE_Theta_pend).*sin(THE_Phi_pend)+cos(THE_Theta).*cos(THE_Phi_pend).*cos(THE_Theta_pend).*sin(THE_Phi)-cos(THE_Psi).*sin(THE_Phi).*sin(THE_Theta).*sin(THE_Theta_pend)+cos(THE_Theta_pend).*sin(THE_Phi).*sin(THE_Psi).*sin(THE_Theta).*sin(THE_Phi_pend)))./2.0,Lz_pend.*m_pend.*cos(THE_Psi_pend).*(cos(THE_Psi).*cos(THE_Theta).*sin(THE_Theta_pend)+cos(THE_Phi_pend).*cos(THE_Theta_pend).*sin(THE_Theta)-cos(THE_Theta).*cos(THE_Theta_pend).*sin(THE_Psi).*sin(THE_Phi_pend)).*(-1.0./2.0),m_pend.*cos(THE_Psi_pend).*cos(THE_Theta_pend).*sin(THE_Psi_pend).*(Ly_pend.^2-Lz_pend.^2.*4.0).*(-1.0./1.2e+1),(m_pend.*(Ly_pend.^2.*sin(THE_Psi_pend).^2-Lz_pend.^2.*sin(THE_Psi_pend).^2.*4.0+Lx_pend.^2+Lz_pend.^2.*4.0))./1.2e+1,0.0,Ly_pend.^2.*m_pend.*cos(THE_Psi).*cos(THE_Theta).*sin(THE_Theta_pend).*(-1.0./1.2e+1)-(Ly_pend.^2.*m_pend.*cos(THE_Phi_pend).*cos(THE_Theta_pend).*sin(THE_Theta))./1.2e+1-(Lz_pend.^2.*m_pend.*cos(THE_Psi).*cos(THE_Theta).*sin(THE_Theta_pend))./3.0-(Lz_pend.^2.*m_pend.*cos(THE_Phi_pend).*cos(THE_Theta_pend).*sin(THE_Theta))./3.0+(Ly_pend.^2.*m_pend.*cos(THE_Theta).*cos(THE_Theta_pend).*sin(THE_Psi).*sin(THE_Phi_pend))./1.2e+1+(Lz_pend.^2.*m_pend.*cos(THE_Theta).*cos(THE_Theta_pend).*sin(THE_Psi).*sin(THE_Phi_pend))./3.0-(Lz_pend.*Tv_Z_pend.*m_pend.*cos(THE_Phi_pend).*cos(THE_Psi_pend).*sin(THE_Theta))./2.0+(Lz_pend.*Tv_Z_pend.*m_pend.*cos(THE_Theta).*cos(THE_Psi_pend).*sin(THE_Psi).*sin(THE_Phi_pend))./2.0-(Lz_pend.*Tv_Z_pend.*m_pend.*sin(THE_Theta).*sin(THE_Phi_pend).*sin(THE_Psi_pend).*sin(THE_Theta_pend))./2.0-(Lz_pend.*Tv_Z_pend.*m_pend.*cos(THE_Theta).*cos(THE_Phi_pend).*sin(THE_Psi).*sin(THE_Psi_pend).*sin(THE_Theta_pend))./2.0,(Ly_pend.^2.*m_pend.*sin(THE_Psi).*sin(THE_Theta_pend))./1.2e+1+(Lz_pend.^2.*m_pend.*sin(THE_Psi).*sin(THE_Theta_pend))./3.0+(Ly_pend.^2.*m_pend.*cos(THE_Psi).*cos(THE_Theta_pend).*sin(THE_Phi_pend))./1.2e+1+(Lz_pend.^2.*m_pend.*cos(THE_Psi).*cos(THE_Theta_pend).*sin(THE_Phi_pend))./3.0+(Lz_pend.*Tv_Z_pend.*m_pend.*cos(THE_Psi).*cos(THE_Psi_pend).*sin(THE_Phi_pend))./2.0-(Lz_pend.*Tv_Z_pend.*m_pend.*cos(THE_Psi).*cos(THE_Phi_pend).*sin(THE_Psi_pend).*sin(THE_Theta_pend))./2.0,(m_pend.*(Ly_pend.^2.*cos(THE_Phi_pend).*cos(THE_Theta_pend)+Lz_pend.^2.*cos(THE_Phi_pend).*cos(THE_Theta_pend).*4.0+Lz_pend.*Tv_Z_pend.*cos(THE_Phi_pend).*cos(THE_Psi_pend).*6.0+Lz_pend.*Tv_Z_pend.*sin(THE_Phi_pend).*sin(THE_Psi_pend).*sin(THE_Theta_pend).*6.0))./1.2e+1,Lz_pend.*m_pend.*(-cos(THE_Psi).*cos(THE_Phi_pend).*cos(THE_Psi_pend).*sin(THE_Phi)-cos(THE_Phi).*cos(THE_Theta).*cos(THE_Psi_pend).*sin(THE_Phi_pend)+cos(THE_Theta_pend).*sin(THE_Phi).*sin(THE_Psi).*sin(THE_Psi_pend)+cos(THE_Phi).*cos(THE_Phi_pend).*cos(THE_Psi_pend).*sin(THE_Psi).*sin(THE_Theta)+cos(THE_Phi).*cos(THE_Psi).*cos(THE_Theta_pend).*sin(THE_Theta).*sin(THE_Psi_pend)+cos(THE_Phi).*cos(THE_Theta).*cos(THE_Phi_pend).*sin(THE_Psi_pend).*sin(THE_Theta_pend)-cos(THE_Psi).*sin(THE_Phi).*sin(THE_Phi_pend).*sin(THE_Psi_pend).*sin(THE_Theta_pend)+cos(THE_Phi).*sin(THE_Psi).*sin(THE_Theta).*sin(THE_Phi_pend).*sin(THE_Psi_pend).*sin(THE_Theta_pend)).*(-1.0./2.0),Lz_pend.*m_pend.*(cos(THE_Phi).*cos(THE_Psi).*cos(THE_Phi_pend).*cos(THE_Psi_pend)-cos(THE_Theta).*cos(THE_Psi_pend).*sin(THE_Phi).*sin(THE_Phi_pend)-cos(THE_Phi).*cos(THE_Theta_pend).*sin(THE_Psi).*sin(THE_Psi_pend)+cos(THE_Phi_pend).*cos(THE_Psi_pend).*sin(THE_Phi).*sin(THE_Psi).*sin(THE_Theta)+cos(THE_Psi).*cos(THE_Theta_pend).*sin(THE_Phi).*sin(THE_Theta).*sin(THE_Psi_pend)+cos(THE_Phi).*cos(THE_Psi).*sin(THE_Phi_pend).*sin(THE_Psi_pend).*sin(THE_Theta_pend)+cos(THE_Theta).*cos(THE_Phi_pend).*sin(THE_Phi).*sin(THE_Psi_pend).*sin(THE_Theta_pend)+sin(THE_Phi).*sin(THE_Psi).*sin(THE_Theta).*sin(THE_Phi_pend).*sin(THE_Psi_pend).*sin(THE_Theta_pend)).*(-1.0./2.0),Lz_pend.*m_pend.*(cos(THE_Psi_pend).*sin(THE_Theta).*sin(THE_Phi_pend)+cos(THE_Theta).*cos(THE_Phi_pend).*cos(THE_Psi_pend).*sin(THE_Psi)+cos(THE_Psi).*cos(THE_Theta).*cos(THE_Theta_pend).*sin(THE_Psi_pend)-cos(THE_Phi_pend).*sin(THE_Theta).*sin(THE_Psi_pend).*sin(THE_Theta_pend)+cos(THE_Theta).*sin(THE_Psi).*sin(THE_Phi_pend).*sin(THE_Psi_pend).*sin(THE_Theta_pend)).*(-1.0./2.0),m_pend.*sin(THE_Theta_pend).*(Ly_pend.^2+Lz_pend.^2.*4.0).*(-1.0./1.2e+1),0.0,(m_pend.*(Ly_pend.^2+Lz_pend.^2.*4.0))./1.2e+1],[9,9]);
if nargout > 1
